simulink library "autolibshared"  (R2019b)
settings: Solver=ode45  StartTime=0.0  StopTime=10.0  RelTol=1e-3  EnableMultiTasking=on
undefined symbols (not defined in the file or in its folder): AccelCycle, aMode, DriveCycle, GearCycle, psi, x_o
libraries: autolibsharedcommon x20, $bdroot x7, autolibutils x2, autolibpowerinfoutils x1
(part 1 of 4)
Description:
  | Automotive Blockset Library: Shared Blocks
settings Model: ModifiedByFormat=The MathWorks, Inc.  Creator=The MathWorks, Inc.  LastModifiedBy=The MathWorks, Inc.
settings SolverCC: MinimalZcImpactIntegration=on
settings DataIOCC: LimitDataPoints=on  SaveFormat=Array  ReturnWorkspaceOutputs=off
settings OptimizationCC: LifeSpan=inf
settings DebuggingCC: SolverPrmCheckMsg=warning  AllowSymbolicDim=off  PregeneratedLibrarySubsystemCodeDiagnostic=none  SFUnexpectedBacktrackingDiag=warning  SFNoUnconditionalDefaultTransitionDiag=warning  SFExecutionAtInitializationDiag=none  ArithmeticOperatorsInVariantConditions=warning
settings ModelReferenceCC: PropagateSignalLabelsOutOfModel=off
settings SFSimCC: SimUseLocalCustomCode=off  CustomCodeUndefinedFunction=UseInterfaceOnly
settings RTWCC: RTWUseLocalCustomCode=off
settings CodeAppCC: StateflowObjectComments=on
settings GRTTargetCC: TargetLangStandard=C89/C90 (ANSI)  GeneratePreprocessorConditionals=Disable all
settings ConfigComp: CovMetricSettings=dw  CovHtmlReporting=on  CovSaveCumulativeToWorkspaceVar=on  CovSaveSingleToWorkspaceVar=on  CovShowResultsExplorer=off  CovExternalEMLEnable=off  CovSFcnEnable=off

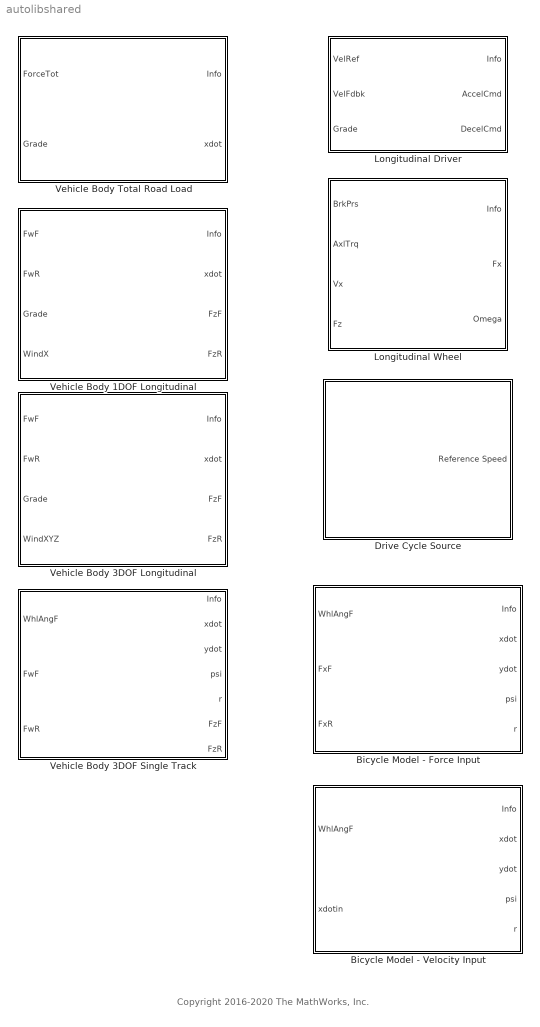
== system autolibshared ==
  note: Copyright 2016-2020 The MathWorks, Inc.
  Bicycle Model - Force Input : Subsystem  mask(Vehicle Body 3DOF Lateral){trackMode=Single (bicycle), inputMode=External longitudinal forces, frontSteerMode=on, rearSteerMode=off, windMode=off, muMode=off, extFMode=off, extMMode=off, aMode=aMode, NF=2, NR=2, m=2000, a=1.4, b=1.6, h=0.35, X_o=0, xdot_o=0, CalphaMode=off, sigmaMode=on, w=[1.4,1.4], Cy_f=12e3, Cy_r=11e3, sigma_f=.1, sigma_r=.1, alpha_f_brk=[-.1 .1], Cy_f_data=[-9e3 9e3], alpha_r_brk=[-.1 .1], Cy_r_data=[-9e3 9e3], Y_o=0, ydot_o=0, Izz=4000, psi_o=0, r_o=0, Af=2, Cd=.3, Cl=.1, Cpm=.1, beta_w=[0:0.01:0.3], Cs=[0:0.03:0.9], Cym=[0:0.01:0.3], Pabs=101325, Tair=273, g=9.81, mu=1, xdot_tol=.01, Fznom=5000, Fxtire_sat=1e6, Fytire_sat=1e6, longOff=0, latOff=0, vertOff=0}
      mask prompts: trackMode "autoblks_shared:autoblkVehBody3DofADTF:blkPrm_trackMode"; inputMode "autoblks_shared:autoblkVehBody3DofADTF:blkPrm_inputMode"; frontSteerMode "autoblks_shared:autoblkVehBody3DofADTF:blkPrm_frontSteerMode"; rearSteerMode "autoblks_shared:autoblkVehBody3DofADTF:blkPrm_rearSteerMode"; windMode "autoblks_shared:autoblkVehBody3DofADTF:blkPrm_windMode"; muMode "autoblks_shared:autoblkVehBody3DofADTF:blkPrm_muMode"; extFMode "autoblks_shared:autoblkVehBody3DofADTF:blkPrm_extFMode"; extMMode "autoblks_shared:autoblkVehBody3DofADTF:blkPrm_extMMode"; NF "autoblks_shared:autoblkVehBody3DofADTF:blkPrm_NF"; NR "autoblks_shared:autoblkVehBody3DofADTF:blkPrm_NR"; m "autoblks_shared:autoblkVehBody3DofADTF:blkPrm_m"; a "autoblks_shared:autoblkVehBody3DofADTF:blkPrm_a"; b "autoblks_shared:autoblkVehBody3DofADTF:blkPrm_b"; h "autoblks_shared:autoblkVehBody3DofADTF:blkPrm_h"; X_o "autoblks_shared:autoblkVehBody3DofADTF:blkPrm_X_o"; xdot_o "autoblks_shared:autoblkVehBody3DofADTF:blkPrm_xdot_o"; CalphaMode "autoblks_shared:autoblkVehBody3DofADTF:blkPrm_CalphaMode"; sigmaMode "autoblks_shared:autoblkVehBody3DofADTF:blkPrm_sigmaMode"; w "autoblks_shared:autoblkVehBody3DofADTF:blkPrm_w"; Cy_f "autoblks_shared:autoblkVehBody3DofADTF:blkPrm_Cy_f"; Cy_r "autoblks_shared:autoblkVehBody3DofADTF:blkPrm_Cy_r"; sigma_f "autoblks_shared:autoblkVehBody3DofADTF:blkPrm_sigma_f"; sigma_r "autoblks_shared:autoblkVehBody3DofADTF:blkPrm_sigma_r"; alpha_f_brk "autoblks_shared:autoblkVehBody3DofADTF:blkPrm_alpha_f_brk"; Cy_f_data "autoblks_shared:autoblkVehBody3DofADTF:blkPrm_Cy_f_data"; alpha_r_brk "autoblks_shared:autoblkVehBody3DofADTF:blkPrm_alpha_r_brk"; Cy_r_data "autoblks_shared:autoblkVehBody3DofADTF:blkPrm_Cy_r_data"; Y_o "autoblks_shared:autoblkVehBody3DofADTF:blkPrm_Y_o"; ydot_o "autoblks_shared:autoblkVehBody3DofADTF:blkPrm_ydot_o"; Izz "autoblks_shared:autoblkVehBody3DofADTF:blkPrm_Izz"; psi_o "autoblks_shared:autoblkVehBody3DofADTF:blkPrm_psi_o"; r_o "autoblks_shared:autoblkVehBody3DofADTF:blkPrm_r_o"; Af "autoblks_shared:autoblkVehBody3DofADTF:blkPrm_Af"; Cd "autoblks_shared:autoblkVehBody3DofADTF:blkPrm_Cd"; Cl "autoblks_shared:autoblkVehBody3DofADTF:blkPrm_Cl"; Cpm "autoblks_shared:autoblkVehBody3DofADTF:blkPrm_Cpm"; beta_w "autoblks_shared:autoblkVehBody3DofADTF:blkPrm_beta_w"; Cs "autoblks_shared:autoblkVehBody3DofADTF:blkPrm_Cs"; Cym "autoblks_shared:autoblkVehBody3DofADTF:blkPrm_Cym"; Pabs "autoblks_shared:autoblkVehBody3DofADTF:blkPrm_Pabs"; Tair "autoblks_shared:autoblkVehBody3DofADTF:blkPrm_Tair"; g "autoblks_shared:autoblkVehBody3DofADTF:blkPrm_g"; mu "autoblks_shared:autoblkVehBody3DofADTF:blkPrm_mu"; xdot_tol "autoblks_shared:autoblkVehBody3DofADTF:blkPrm_xdot_tol"; Fznom "autoblks_shared:autoblkVehBody3DofADTF:blkPrm_Fznom"; Fxtire_sat "autoblks_shared:autoblkVehBody3DofADTF:blkPrm_Fxtire_sat"; Fytire_sat "autoblks_shared:autoblkVehBody3DofADTF:blkPrm_Fytire_sat"; longOff "autoblks_shared:autoblkVehBody3DofADTF:blkPrm_longOff"; latOff "autoblks_shared:autoblkVehBody3DofADTF:blkPrm_latOff"; vertOff "autoblks_shared:autoblkVehBody3DofADTF:blkPrm_vertOff"
      mask help: autoblks_shared:autoblkVehBody3DofADTF:blkDesc
      mask init:
      | [~]=autosharedicon('autolibvehdyn3doflatr',gcb,0);
      mask Help: eval('autosharedhelp(''vbbicycle'')');
      mask TypeOptions trackMode: autoblks_shared:autoblkVehBody3DofADTF:blkCmb_trackMode_c1 | autoblks_shared:autoblkVehBody3DofADTF:blkCmb_trackMode_c2
      mask Callback trackMode: %[~]=vehdynicon('vehdynliblat3dof',gcb,5);
      mask TypeOptions inputMode: autoblks_shared:autoblkVehBody3DofADTF:blkCmb_inputMode_c1 | autoblks_shared:autoblkVehBody3DofADTF:blkCmb_inputMode_c2 | autoblks_shared:autoblkVehBody3DofADTF:blkCmb_inputMode_c3
      mask Callback inputMode: %[~]=vehdynicon('vehdynliblat3dof',gcb,1);
      mask Callback muMode: %[~]=vehdynicon('vehdynliblat3dof',gcb,2);
      mask Callback CalphaMode: %[~]=vehdynicon('vehdynliblat3dof',gcb,3);
      mask Callback sigmaMode: %[~]=vehdynicon('vehdynliblat3dof',gcb,4);
      mask TypeOptions longOff: Vehicle Body 3DOF Single Track/longOff
      mask TypeOptions latOff: Vehicle Body 3DOF Single Track/latOff
      mask TypeOptions vertOff: Vehicle Body 3DOF Single Track/vertOff
      mask DialogControl blockConfig Prompt: autoblks_shared:autoblkVehBody3DofADTF:blkDlg_blockConfig
      mask DialogControl trackMode Prompt: Vehicle track:
      mask DialogControl inputMode Prompt: Axle forces:
      mask DialogControl frontSteerMode Prompt: Front wheel steering
      mask DialogControl rearSteerMode Prompt: Rear wheel steering
      mask DialogControl windMode Prompt: External wind
      mask DialogControl muMode Prompt: External friction
      mask DialogControl extFMode Prompt: External forces
      mask DialogControl extMMode Prompt: External moments
      mask DialogControl ParameterGroupVar Prompt: autoblks_shared:autoblkVehBody3DofADTF:blkDlg_ParameterGroupVar
      mask DialogControl LongPanel Prompt: autoblks_shared:autoblkVehBody3DofADTF:blkDlg_LongPanel
      mask DialogControl NF Prompt: Number of wheels on front axle, NF [-]:
      mask DialogControl NR Prompt: Number of wheels on rear axle, NR [-]:
      mask DialogControl m Prompt: Vehicle mass, m [kg]:
      mask DialogControl a Prompt: Longitudinal distance from center of mass to front axle, a [m]:
      mask DialogControl b Prompt: Longitudinal distance from center of mass to rear axle, b [m]:
      mask DialogControl h Prompt: Vertical distance from center of mass to axle plane, h [m]:
      mask DialogControl X_o Prompt: Initial inertial frame longitudinal position, X_o [m]:
      mask DialogControl xdot_o Prompt: Initial longitudinal velocity, xdot_o [m/s]:
      mask DialogControl LatPanel Prompt: autoblks_shared:autoblkVehBody3DofADTF:blkDlg_LatPanel
      mask DialogControl CalphaMode Prompt: Mapped corner stiffness:
      mask DialogControl sigmaMode Prompt: Include relaxation length dynamics:
      mask DialogControl w Prompt: Track width, w [m]:
      mask DialogControl Cy_f Prompt: Front tire corner stiffness, Cy_f [N/rad]:
      mask DialogControl Cy_r Prompt: Rear tire axle corner stiffness, Cy_r [N/rad]:
      mask DialogControl sigma_f Prompt: Front tire(s) relaxation length, sigma_f [m]:
      mask DialogControl sigma_r Prompt: Rear tire(s) relaxation length, sigma_r [m]:
      mask DialogControl alpha_f_brk Prompt: Front axle slip angle breakpoints, alpha_f_brk [rad]:
      mask DialogControl Cy_f_data Prompt: Front axle corner data, Cy_f_data [N/rad]:
      mask DialogControl alpha_r_brk Prompt: Rear axle slip angle breakpoints, alpha_r_brk [rad]:
      mask DialogControl Cy_r_data Prompt: Rear axle corner data, Cy_r_data [N/rad]:
      mask DialogControl Y_o Prompt: Initial inertial frame lateral displacement, Y_o [m]:
      mask DialogControl ydot_o Prompt: Initial lateral velocity, ydot_o [m/s]:
      mask DialogControl YawPanel Prompt: autoblks_shared:autoblkVehBody3DofADTF:blkDlg_YawPanel
      mask DialogControl Izz Prompt: Yaw polar inertia, Izz [kg*m^2]:
      mask DialogControl psi_o Prompt: Initial yaw angle, psi_o [rad]:
      mask DialogControl r_o Prompt: Initial yaw rate, r_o [rad/s]:
      mask DialogControl AeroParams Prompt: autoblks_shared:autoblkVehBody3DofADTF:blkDlg_AeroParams
      mask DialogControl Af Prompt: Longitudinal drag area, Af [m^2]:
      mask DialogControl Cd Prompt: Longitudinal drag coefficient, Cd [-]:
      mask DialogControl Cl Prompt: Longitudinal lift coefficient, Cl [-]:
      mask DialogControl Cpm Prompt: Longitudinal drag pitch moment, Cpm [-]:
      mask DialogControl beta_w Prompt: Relative wind angle vector, beta_w [rad]:
      mask DialogControl Cs Prompt: Side force coefficient vector, Cs [-]:
      mask DialogControl Cym Prompt: Yaw moment coefficient vector, Cym [-]:
      mask DialogControl EnviroPanel Prompt: autoblks_shared:autoblkVehBody3DofADTF:blkDlg_EnviroPanel
      mask DialogControl Pabs Prompt: Absolute pressure, Pabs [Pa]:
      mask DialogControl Tair Prompt: Air temperature, Tair [K]:
      mask DialogControl g Prompt: Gravitational acceleration, g [m/s^2]:
      mask DialogControl mu Prompt: Nominal friction scaling factor, mu [-]:
      mask DialogControl SimPanel Prompt: autoblks_shared:autoblkVehBody3DofADTF:blkDlg_SimPanel
      mask DialogControl xdot_tol Prompt: Longitudinal velocity tolerance, xdot_tol [m/s]:
      mask DialogControl Fznom Prompt: Nominal normal force, Fznom [N]:
      mask DialogControl Fxtire_sat Prompt: Longitudinal force limit, Fxtire_sat [N]:
      mask DialogControl Fytire_sat Prompt: Lateral force limit, Fytire_sat [N]:
      mask DialogControl longOff Prompt: Geometric longitudinal offset from axle plane, longOff [m]:
      mask DialogControl latOff Prompt: Geometric lateral offset from axle plane, latOff [m]:
      mask DialogControl vertOff Prompt: Geometric vertical offset from axle plane, vertOff [m]:
      mask Display:
      | try
      |     IconInfo = autosharedicon('autolibvehdyn3doflatr',gcb,8);
      | 
      |     image(IconInfo.image, IconInfo.position);
      | 
      |     for i = 1:numel(IconInfo.lconn)
      |         port_label('lconn', i, IconInfo.lconn{i})
      |     end
      | 
      |     for j = 1:numel(IconInfo.rconn)
      |         port_label('rconn', j, IconInfo.rconn{j})
      |     end
      | 
      |     for k = 1:numel(IconInfo.input)
      |         port_label('input', k, IconInfo.input{k})
      |     end
      | 
      |     for m = 1:numel(IconInfo.output)
      |         port_label('output', m, IconInfo.output{m})
      |     end
      | catch
      |     fprintf('Vehicle Body \n 3DOF Lateral')
      | end
  Bicycle Model - Velocity Input : Subsystem  mask(Vehicle Body 3DOF Lateral){trackMode=Single (bicycle), inputMode=External longitudinal velocity, frontSteerMode=on, rearSteerMode=off, windMode=off, muMode=off, extFMode=off, extMMode=off, aMode=aMode, NF=2, NR=2, m=2000, a=1.4, b=1.6, h=0.35, X_o=0, xdot_o=0, CalphaMode=off, sigmaMode=on, w=[1.4,1.4], Cy_f=12e3, Cy_r=11e3, sigma_f=.1, sigma_r=.1, alpha_f_brk=[-.1 .1], Cy_f_data=[-9e3 9e3], alpha_r_brk=[-.1 .1], Cy_r_data=[-9e3 9e3], Y_o=0, ydot_o=0, Izz=4000, psi_o=0, r_o=0, Af=2, Cd=.3, Cl=.1, Cpm=.1, beta_w=[0:0.01:0.3], Cs=[0:0.03:0.9], Cym=[0:0.01:0.3], Pabs=101325, Tair=273, g=9.81, mu=1, xdot_tol=.01, Fznom=5000, Fxtire_sat=1e6, Fytire_sat=1e6, longOff=0, latOff=0, vertOff=0}
      mask prompts: trackMode "autoblks_shared:autoblkVehBody3DofADTx:blkPrm_trackMode"; inputMode "autoblks_shared:autoblkVehBody3DofADTx:blkPrm_inputMode"; frontSteerMode "autoblks_shared:autoblkVehBody3DofADTx:blkPrm_frontSteerMode"; rearSteerMode "autoblks_shared:autoblkVehBody3DofADTx:blkPrm_rearSteerMode"; windMode "autoblks_shared:autoblkVehBody3DofADTx:blkPrm_windMode"; muMode "autoblks_shared:autoblkVehBody3DofADTx:blkPrm_muMode"; extFMode "autoblks_shared:autoblkVehBody3DofADTx:blkPrm_extFMode"; extMMode "autoblks_shared:autoblkVehBody3DofADTx:blkPrm_extMMode"; NF "autoblks_shared:autoblkVehBody3DofADTx:blkPrm_NF"; NR "autoblks_shared:autoblkVehBody3DofADTx:blkPrm_NR"; m "autoblks_shared:autoblkVehBody3DofADTx:blkPrm_m"; a "autoblks_shared:autoblkVehBody3DofADTx:blkPrm_a"; b "autoblks_shared:autoblkVehBody3DofADTx:blkPrm_b"; h "autoblks_shared:autoblkVehBody3DofADTx:blkPrm_h"; X_o "autoblks_shared:autoblkVehBody3DofADTx:blkPrm_X_o"; xdot_o "autoblks_shared:autoblkVehBody3DofADTx:blkPrm_xdot_o"; CalphaMode "autoblks_shared:autoblkVehBody3DofADTx:blkPrm_CalphaMode"; sigmaMode "autoblks_shared:autoblkVehBody3DofADTx:blkPrm_sigmaMode"; w "autoblks_shared:autoblkVehBody3DofADTx:blkPrm_w"; Cy_f "autoblks_shared:autoblkVehBody3DofADTx:blkPrm_Cy_f"; Cy_r "autoblks_shared:autoblkVehBody3DofADTx:blkPrm_Cy_r"; sigma_f "autoblks_shared:autoblkVehBody3DofADTx:blkPrm_sigma_f"; sigma_r "autoblks_shared:autoblkVehBody3DofADTx:blkPrm_sigma_r"; alpha_f_brk "autoblks_shared:autoblkVehBody3DofADTx:blkPrm_alpha_f_brk"; Cy_f_data "autoblks_shared:autoblkVehBody3DofADTx:blkPrm_Cy_f_data"; alpha_r_brk "autoblks_shared:autoblkVehBody3DofADTx:blkPrm_alpha_r_brk"; Cy_r_data "autoblks_shared:autoblkVehBody3DofADTx:blkPrm_Cy_r_data"; Y_o "autoblks_shared:autoblkVehBody3DofADTx:blkPrm_Y_o"; ydot_o "autoblks_shared:autoblkVehBody3DofADTx:blkPrm_ydot_o"; Izz "autoblks_shared:autoblkVehBody3DofADTx:blkPrm_Izz"; psi_o "autoblks_shared:autoblkVehBody3DofADTx:blkPrm_psi_o"; r_o "autoblks_shared:autoblkVehBody3DofADTx:blkPrm_r_o"; Af "autoblks_shared:autoblkVehBody3DofADTx:blkPrm_Af"; Cd "autoblks_shared:autoblkVehBody3DofADTx:blkPrm_Cd"; Cl "autoblks_shared:autoblkVehBody3DofADTx:blkPrm_Cl"; Cpm "autoblks_shared:autoblkVehBody3DofADTx:blkPrm_Cpm"; beta_w "autoblks_shared:autoblkVehBody3DofADTx:blkPrm_beta_w"; Cs "autoblks_shared:autoblkVehBody3DofADTx:blkPrm_Cs"; Cym "autoblks_shared:autoblkVehBody3DofADTx:blkPrm_Cym"; Pabs "autoblks_shared:autoblkVehBody3DofADTx:blkPrm_Pabs"; Tair "autoblks_shared:autoblkVehBody3DofADTx:blkPrm_Tair"; g "autoblks_shared:autoblkVehBody3DofADTx:blkPrm_g"; mu "autoblks_shared:autoblkVehBody3DofADTx:blkPrm_mu"; xdot_tol "autoblks_shared:autoblkVehBody3DofADTx:blkPrm_xdot_tol"; Fznom "autoblks_shared:autoblkVehBody3DofADTx:blkPrm_Fznom"; Fxtire_sat "autoblks_shared:autoblkVehBody3DofADTx:blkPrm_Fxtire_sat"; Fytire_sat "autoblks_shared:autoblkVehBody3DofADTx:blkPrm_Fytire_sat"; longOff "autoblks_shared:autoblkVehBody3DofADTx:blkPrm_longOff"; latOff "autoblks_shared:autoblkVehBody3DofADTx:blkPrm_latOff"; vertOff "autoblks_shared:autoblkVehBody3DofADTx:blkPrm_vertOff"
      mask help: autoblks_shared:autoblkVehBody3DofADTx:blkDesc
      mask init:
      | [~]=autosharedicon('autolibvehdyn3doflatr',gcb,0);
      mask Help: eval('autosharedhelp(''vbbicycle'')');
      mask TypeOptions trackMode: autoblks_shared:autoblkVehBody3DofADTx:blkCmb_trackMode_c1 | autoblks_shared:autoblkVehBody3DofADTx:blkCmb_trackMode_c2
      mask Callback trackMode: %[~]=vehdynicon('vehdynliblat3dof',gcb,5);
      mask TypeOptions inputMode: autoblks_shared:autoblkVehBody3DofADTx:blkCmb_inputMode_c1 | autoblks_shared:autoblkVehBody3DofADTx:blkCmb_inputMode_c2 | autoblks_shared:autoblkVehBody3DofADTx:blkCmb_inputMode_c3
      mask Callback inputMode: %[~]=vehdynicon('vehdynliblat3dof',gcb,1);
      mask Callback muMode: %[~]=vehdynicon('vehdynliblat3dof',gcb,2);
      mask Callback CalphaMode: %[~]=vehdynicon('vehdynliblat3dof',gcb,3);
      mask Callback sigmaMode: %[~]=vehdynicon('vehdynliblat3dof',gcb,4);
      mask TypeOptions longOff: Vehicle Body 3DOF Single Track/longOff
      mask TypeOptions latOff: Vehicle Body 3DOF Single Track/latOff
      mask TypeOptions vertOff: Vehicle Body 3DOF Single Track/vertOff
      mask DialogControl blockConfig Prompt: autoblks_shared:autoblkVehBody3DofADTx:blkDlg_blockConfig
      mask DialogControl trackMode Prompt: Vehicle track:
      mask DialogControl inputMode Prompt: Axle forces:
      mask DialogControl frontSteerMode Prompt: Front wheel steering
      mask DialogControl rearSteerMode Prompt: Rear wheel steering
      mask DialogControl windMode Prompt: External wind
      mask DialogControl muMode Prompt: External friction
      mask DialogControl extFMode Prompt: External forces
      mask DialogControl extMMode Prompt: External moments
      mask DialogControl ParameterGroupVar Prompt: autoblks_shared:autoblkVehBody3DofADTx:blkDlg_ParameterGroupVar
      mask DialogControl LongPanel Prompt: autoblks_shared:autoblkVehBody3DofADTx:blkDlg_LongPanel
      mask DialogControl NF Prompt: Number of wheels on front axle, NF [-]:
      mask DialogControl NR Prompt: Number of wheels on rear axle, NR [-]:
      mask DialogControl m Prompt: Vehicle mass, m [kg]:
      mask DialogControl a Prompt: Longitudinal distance from center of mass to front axle, a [m]:
      mask DialogControl b Prompt: Longitudinal distance from center of mass to rear axle, b [m]:
      mask DialogControl h Prompt: Vertical distance from center of mass to axle plane, h [m]:
      mask DialogControl X_o Prompt: Initial inertial frame longitudinal position, X_o [m]:
      mask DialogControl xdot_o Prompt: Initial longitudinal velocity, xdot_o [m/s]:
      mask DialogControl LatPanel Prompt: autoblks_shared:autoblkVehBody3DofADTx:blkDlg_LatPanel
      mask DialogControl CalphaMode Prompt: Mapped corner stiffness:
      mask DialogControl sigmaMode Prompt: Include relaxation length dynamics:
      mask DialogControl w Prompt: Track width, w [m]:
      mask DialogControl Cy_f Prompt: Front tire corner stiffness, Cy_f [N/rad]:
      mask DialogControl Cy_r Prompt: Rear tire axle corner stiffness, Cy_r [N/rad]:
      mask DialogControl sigma_f Prompt: Front tire(s) relaxation length, sigma_f [m]:
      mask DialogControl sigma_r Prompt: Rear tire(s) relaxation length, sigma_r [m]:
      mask DialogControl alpha_f_brk Prompt: Front axle slip angle breakpoints, alpha_f_brk [rad]:
      mask DialogControl Cy_f_data Prompt: Front axle corner data, Cy_f_data [N/rad]:
      mask DialogControl alpha_r_brk Prompt: Rear axle slip angle breakpoints, alpha_r_brk [rad]:
      mask DialogControl Cy_r_data Prompt: Rear axle corner data, Cy_r_data [N/rad]:
      mask DialogControl Y_o Prompt: Initial inertial frame lateral displacement, Y_o [m]:
      mask DialogControl ydot_o Prompt: Initial lateral velocity, ydot_o [m/s]:
      mask DialogControl YawPanel Prompt: autoblks_shared:autoblkVehBody3DofADTx:blkDlg_YawPanel
      mask DialogControl Izz Prompt: Yaw polar inertia, Izz [kg*m^2]:
      mask DialogControl psi_o Prompt: Initial yaw angle, psi_o [rad]:
      mask DialogControl r_o Prompt: Initial yaw rate, r_o [rad/s]:
      mask DialogControl AeroParams Prompt: autoblks_shared:autoblkVehBody3DofADTx:blkDlg_AeroParams
      mask DialogControl Af Prompt: Longitudinal drag area, Af [m^2]:
      mask DialogControl Cd Prompt: Longitudinal drag coefficient, Cd [-]:
      mask DialogControl Cl Prompt: Longitudinal lift coefficient, Cl [-]:
      mask DialogControl Cpm Prompt: Longitudinal drag pitch moment, Cpm [-]:
      mask DialogControl beta_w Prompt: Relative wind angle vector, beta_w [rad]:
      mask DialogControl Cs Prompt: Side force coefficient vector, Cs [-]:
      mask DialogControl Cym Prompt: Yaw moment coefficient vector, Cym [-]:
      mask DialogControl EnviroPanel Prompt: autoblks_shared:autoblkVehBody3DofADTx:blkDlg_EnviroPanel
      mask DialogControl Pabs Prompt: Absolute pressure, Pabs [Pa]:
      mask DialogControl Tair Prompt: Air temperature, Tair [K]:
      mask DialogControl g Prompt: Gravitational acceleration, g [m/s^2]:
      mask DialogControl mu Prompt: Nominal friction scaling factor, mu [-]:
      mask DialogControl SimPanel Prompt: autoblks_shared:autoblkVehBody3DofADTx:blkDlg_SimPanel
      mask DialogControl xdot_tol Prompt: Longitudinal velocity tolerance, xdot_tol [m/s]:
      mask DialogControl Fznom Prompt: Nominal normal force, Fznom [N]:
      mask DialogControl Fxtire_sat Prompt: Longitudinal force limit, Fxtire_sat [N]:
      mask DialogControl Fytire_sat Prompt: Lateral force limit, Fytire_sat [N]:
      mask DialogControl longOff Prompt: Geometric longitudinal offset from axle plane, longOff [m]:
      mask DialogControl latOff Prompt: Geometric lateral offset from axle plane, latOff [m]:
      mask DialogControl vertOff Prompt: Geometric vertical offset from axle plane, vertOff [m]:
      mask Display:
      | try
      |     IconInfo = autosharedicon('autolibvehdyn3doflatr',gcb,8);
      | 
      |     image(IconInfo.image, IconInfo.position);
      | 
      |     for i = 1:numel(IconInfo.lconn)
      |         port_label('lconn', i, IconInfo.lconn{i})
      |     end
      | 
      |     for j = 1:numel(IconInfo.rconn)
      |         port_label('rconn', j, IconInfo.rconn{j})
      |     end
      | 
      |     for k = 1:numel(IconInfo.input)
      |         port_label('input', k, IconInfo.input{k})
      |     end
      | 
      |     for m = 1:numel(IconInfo.output)
      |         port_label('output', m, IconInfo.output{m})
      |     end
      | catch
      |     fprintf('Vehicle Body \n 3DOF Lateral')
      | end
  Drive Cycle Source : Subsystem  mask(Drive Cycle Source){cycleVar=FTP75, wsVar=, fileVar=cycleFTP75.mat, tfinal=2474  seconds, cycleRepeat=off, outAccPort=off, outGearPort=off, gearList=No gear data, t_wot1=5, xdot_woto=0, xdot_wot1=30, t_wot2=20, xdot_wot2=0, t_wotend=30, srcUnit=m/s, outUnit=m/s, srcAccUnit=m/s/s, outAccUnit=m/s^2, dt=0, aMode=aMode}
      mask prompts: cycleVar "autoblks_shared:autoblkDriveCycleSource:blkPrm_cycleVar"; wsVar "autoblks_shared:autoblkDriveCycleSource:blkPrm_wsVar"; fileVar "autoblks_shared:autoblkDriveCycleSource:blkPrm_fileVar"; tfinal "autoblks_shared:autoblkDriveCycleSource:blkPrm_tfinal"; cycleRepeat "autoblks_shared:autoblkDriveCycleSource:blkPrm_cycleRepeat"; outAccPort "autoblks_shared:autoblkDriveCycleSource:blkPrm_outAccPort"; outGearPort "Output gear shift data"; gearList "Select gear data:"; t_wot1 "autoblks_shared:autoblkDriveCycleSource:blkPrm_t_wot1"; xdot_woto "autoblks_shared:autoblkDriveCycleSource:blkPrm_xdot_woto"; xdot_wot1 "autoblks_shared:autoblkDriveCycleSource:blkPrm_xdot_wot1"; t_wot2 "autoblks_shared:autoblkDriveCycleSource:blkPrm_t_wot2"; xdot_wot2 "autoblks_shared:autoblkDriveCycleSource:blkPrm_xdot_wot2"; t_wotend "autoblks_shared:autoblkDriveCycleSource:blkPrm_t_wotend"; srcUnit "autoblks_shared:autoblkDriveCycleSource:blkPrm_srcUnit"; outUnit "autoblks_shared:autoblkDriveCycleSource:blkPrm_outUnit"; srcAccUnit "autoblks_shared:autoblkDriveCycleSource:blkPrm_srcAccUnit"; outAccUnit "autoblks_shared:autoblkDriveCycleSource:blkPrm_outAccUnit"; dt "autoblks_shared:autoblkDriveCycleSource:blkPrm_dt"
      mask help: autoblks_shared:autoblkDriveCycleSource:blkDesc
      mask init:
      | [DriveCycle, AccelCycle, GearCycle] = autosharedicon('autolibdrivecycle',gcb,0);
      settings: AttributesFormatString=%<cycleVar> (%<tfinal>)
      mask Help: eval('autosharedhelp(''pbdrivecyclelong'')');
      mask TypeOptions cycleVar: FTP72 | FTP75 | US06 | SC03 | HWFET | NYCC | HUDDS | LA92 | LA92Short | IM240 | UDDS | WLTP Class 1 | WLTP Class 2 | WLTP Class 3 | ECE R15 (single cycle) | ECE R15 (four cycles) | EUDC | ECE Extra-Urban Driving Cycle (Low Powered Vehicles) | NEDC | ADAC BAB 130 | Artemis Urban | Artemis Rural Road | Artemis Motorway 130 kmph | Artemis Motorway 150 kmph | JC08 | JC08 Hot | Japanese 10 Mode | Japanese 15 Mode | Japanese 10-15 Mode | World Harmonized Vehicle Cycle (WHVC) | Braunschweig City Driving Cycle | Central Business District (CBD) Cycle | Business Arterial Commuter (BAC) - Arterial Cycle | Business Arterial Commuter (BAC) - Commuter Cycle | City Suburban Heavy Vehicle Cycle (CSC) | Neighborhood Refuse Truck Cycle | New York Composite Cycle | New York Bus Cycle | Manhattan Bus Cycle | Heavy Heavy-Duty Diesel Truck (HHDDT) - Creep Mode | Heavy Heavy-Duty Diesel Truck (HHDDT) - Transient Mode | Heavy Heavy-Duty Diesel Truck (HHDDT) - Cruise Mode | Orange County Bus Cycle | West Virginia University 5-Peak Truck Cycle | RTS 95 | ETC FIGE Version 4 | JE05 Japanese Transient Mode for vehicles > 3500 kg GVW | CUEDC Petrol cycle | CUEDC SPC240 cycle | CUEDC diesel cycle - MC | CUEDC diesel cycle - NA | CUEDC diesel cycle - NB | CUEDC diesel cycle - ME | CUEDC diesel cycle - NC | CUEDC diesel cycle - NCH | Wide Open Throttle (WOT) | Workspace variable | .mat, .xls, .xlsx or .txt file
      mask Callback cycleVar: [~,~] = autosharedicon('autolibdrivecycle',gcb,1);
      mask Callback outAccPort: [~,~] = autosharedicon('autolibdrivecycle',gcb,5);
      mask Callback outGearPort: [~,~] = autosharedicon('autolibdrivecycle',gcb,6);
      mask TypeOptions gearList: No gear data
      mask TypeOptions srcUnit: timing mode/Continuous/Spd/Unit | timing mode/Discrete/Spd/Unit
      mask TypeOptions outUnit: Reference Speed/Unit
      mask TypeOptions srcAccUnit: timing mode/Continuous/Acc/Unit | timing mode/Discrete/Acc/Unit
      mask DialogControl cycleVar Prompt: Drive cycle source:
      mask DialogControl wsVar Prompt: From workspace:
      mask DialogControl fileVar Prompt: Drive cycle source file:
      mask DialogControl wsVarSel Prompt: autoblks_shared:autoblkDriveCycleSource:blkDlg_wsVarSel
      mask DialogControl wsVarSel Callback:
      | set_param(gcb,'cycleVar','Workspace variable');
      | [~,~] = autosharedicon('autolibdrivecycle',gcb,1);
      mask DialogControl fileSel Prompt: autoblks_shared:autoblkDriveCycleSource:blkDlg_fileSel
      mask DialogControl fileSel Callback: [~,~] = autosharedicon('autolibdrivecycle',gcb,2);
      mask DialogControl getData Prompt: autoblks_shared:autoblkDriveCycleSource:blkDlg_getData
      mask DialogControl getData Callback: autoDataPackage(gcb)
      mask DialogControl tfinal Prompt: Total drive cycle time:
      mask DialogControl cycleRepeat Prompt: Repeat cyclically
      mask DialogControl outAccPort Prompt: Output acceleration
      mask DialogControl wotParam Prompt: autoblks_shared:autoblkDriveCycleSource:blkDlg_wotParam
      mask DialogControl t_wot1 Prompt: Start time, t_wot1 [s]:
      mask DialogControl xdot_woto Prompt: Initial reference speed, xdot_woto []:
      mask DialogControl xdot_wot1 Prompt: Nominal reference speed, xdot_wot1 []:
      mask DialogControl t_wot2 Prompt: Time to start deceleration, t_wot2 [s]:
      mask DialogControl xdot_wot2 Prompt: Final reference speed, xdot_wot2 []:
      mask DialogControl t_wotend Prompt: WOT simulation time, t_wotend []:
      mask DialogControl unitsParam Prompt: autoblks_shared:autoblkDriveCycleSource:blkDlg_unitsParam
      mask DialogControl srcUnit Prompt: Source velocity units (e.g., m/s, km/h, mph):
      mask DialogControl outUnit Prompt: Output velocity units (e.g., m/s, km/h, mph):
      mask DialogControl srcAccUnit Prompt: Source acceleration units (e.g., m/s^2, ft/s^2):
      mask DialogControl outAccUnit Prompt: Output acceleration units (e.g., m/s^2, ft/s^2):
      mask DialogControl dt Prompt: Output sample period (0 for continuous), dt [s]:
      mask DialogControl updateSim Prompt: autoblks_shared:autoblkDriveCycleSource:blkDlg_updateSim
      mask DialogControl updateSim Callback: [~,~] = autosharedicon('autolibdrivecycle',gcb,3);
      mask DialogControl plotCycle Prompt: autoblks_shared:autoblkDriveCycleSource:blkDlg_plotCycle
      mask DialogControl plotCycle Callback: [~,~] = autosharedicon('autolibdrivecycle',gcb,4);
      mask Display:
      | try
      |     if exist('DriveCycle','var') && ~isempty(DriveCycle)
      |         plot(DriveCycle.Time./max(DriveCycle.Time).*0.75,DriveCycle.Data./max(DriveCycle.Data))
      |     end
      |     AliasNames = {'Reference Speed','RefSpd';...
      |                   'Reference Accel','RefAcc';...
      |                   'Reference Gear','RefGear'};
      |     IconInfo = autoblksgetportlabels(gcb, AliasNames);
      |     for m = 1:numel(IconInfo.output)
      |         port_label('output', m, IconInfo.output{m})
      |     end
      | catch
      |     fprintf('Drive Cycle Source')
      | end
  Longitudinal Driver : Subsystem  SystemSampleTime=.01  mask(Longitudinal Driver){cntrlType=PI, shftType=None, velUnits=m/s, gearOut=off, Kp=10, Ki=5, Kff=.1, Kg=0, VehVelVec=[0 100], KffVec=[.1 .1], KpVec=[10 10], KiVec=[5 5], KgVec=[0 0], m=1500, Kpt=10000, tau=.2, L=4, aR=200, bR=2.5, cR=.5, g=9.81, vnom=5, Kaw=1, tauerr=.01, tauPt=2, GearInit=0, tShift=.1, pdlVec=[0.1 0.4 0.5 0.9], upShftTbl=[-1 12.9375 26.4375 39.9375 51.18749999999999 62.4375 72.84375 83.25;-1 16.3125 29.8125 43.3125 54.5624 65.8125 76.78125 87.75;-1 19.6875 33.1875 46.68749999999999 57.9375 69.1875 80.71875 92.25;-1 33 52.5 77.25 100.5 138.75 161.875 185], dwnShftTbl=[1 9.5625 23.0625 36.5625 47.8125 59.0625 68.90625 78.75;1 12.9375 26.4375 39.9375 51.18749999999999 62.4375 72.84375 83.25;1 16.3125 29.8125 43.3125 54.562499 65.8125 76.78125 87.75;1 19.6875 33.1875 46.68749999999999 57.9375 69.1875 80.71875 92.25], tClutch=.5, tRev=.5, tPark=120, aMode=aMode, UpGearVec=[0  1  2  3  4  5  6  7], DownGearVec=[1  2  3  4  5  6  7  8]}
      mask prompts: cntrlType "autoblks_shared:autoblkLongitudinalDriver:blkPrm_cntrlType"; shftType "autoblks_shared:autoblkLongitudinalDriver:blkPrm_shftType"; velUnits "autoblks_shared:autoblkLongitudinalDriver:blkPrm_velUnits"; gearOut "autoblks_shared:autoblkLongitudinalDriver:blkPrm_gearOut"; Kp "autoblks_shared:autoblkLongitudinalDriver:blkPrm_Kp"; Ki "autoblks_shared:autoblkLongitudinalDriver:blkPrm_Ki"; Kff "autoblks_shared:autoblkLongitudinalDriver:blkPrm_Kff"; Kg "autoblks_shared:autoblkLongitudinalDriver:blkPrm_Kg"; VehVelVec "autoblks_shared:autoblkLongitudinalDriver:blkPrm_VehVelVec"; KffVec "autoblks_shared:autoblkLongitudinalDriver:blkPrm_KffVec"; KpVec "autoblks_shared:autoblkLongitudinalDriver:blkPrm_KpVec"; KiVec "autoblks_shared:autoblkLongitudinalDriver:blkPrm_KiVec"; KgVec "autoblks_shared:autoblkLongitudinalDriver:blkPrm_KgVec"; m "autoblks_shared:autoblkLongitudinalDriver:blkPrm_m"; Kpt "autoblks_shared:autoblkLongitudinalDriver:blkPrm_Kpt"; tau "autoblks_shared:autoblkLongitudinalDriver:blkPrm_tau"; L "autoblks_shared:autoblkLongitudinalDriver:blkPrm_L"; aR "autoblks_shared:autoblkLongitudinalDriver:blkPrm_aR"; bR "autoblks_shared:autoblkLongitudinalDriver:blkPrm_bR"; cR "autoblks_shared:autoblkLongitudinalDriver:blkPrm_cR"; g "autoblks_shared:autoblkLongitudinalDriver:blkPrm_g"; vnom "autoblks_shared:autoblkLongitudinalDriver:blkPrm_vnom"; Kaw "autoblks_shared:autoblkLongitudinalDriver:blkPrm_Kaw"; tauerr "autoblks_shared:autoblkLongitudinalDriver:blkPrm_tauerr"; tauPt "Powertrain time constant, tauPt [s]:"; GearInit "autoblks_shared:autoblkLongitudinalDriver:blkPrm_GearInit"; tShift "autoblks_shared:autoblkLongitudinalDriver:blkPrm_tShift"; pdlVec "autoblks_shared:autoblkLongitudinalDriver:blkPrm_pdlVec"; upShftTbl "autoblks_shared:autoblkLongitudinalDriver:blkPrm_upShftTbl"; dwnShftTbl "autoblks_shared:autoblkLongitudinalDriver:blkPrm_dwnShftTbl"; tClutch "autoblks_shared:autoblkLongitudinalDriver:blkPrm_tClutch"; tRev "autoblks_shared:autoblkLongitudinalDriver:blkPrm_tRev"; tPark "autoblks_shared:autoblkLongitudinalDriver:blkPrm_tPark"; UpGearVec "autoblks_shared:autoblkLongitudinalDriver:blkPrm_UpGearVec"; DownGearVec "autoblks_shared:autoblkLongitudinalDriver:blkPrm_DownGearVec"
      mask help: autoblks_shared:autoblkLongitudinalDriver:blkDesc
      mask init:
      | [~]=autosharedicon('autoliboperlong',gcb,0);
      mask Help: eval('autosharedhelp(''pbopmodlong'')');
      mask TypeOptions cntrlType: autoblks_shared:autoblkLongitudinalDriver:blkCmb_cntrlType_c1 | autoblks_shared:autoblkLongitudinalDriver:blkCmb_cntrlType_c2 | autoblks_shared:autoblkLongitudinalDriver:blkCmb_cntrlType_c3
      mask Callback cntrlType: [~]=autosharedicon('autoliboperlong',gcb,1);
      mask TypeOptions shftType: Longitudinal Driver/shftType
      mask TypeOptions velUnits: VelRef/Unit
      mask Callback velUnits: [~]=autosharedicon('autoliboperlong',gcb,1);
      mask DialogControl modeConfig Prompt: autoblks_shared:autoblkLongitudinalDriver:blkDlg_modeConfig
      mask DialogControl cntrlType Prompt: Control type, cntrlType:
      mask DialogControl shftType Prompt: Shift type, shftType:
      mask DialogControl velUnits Prompt: Reference and feedback units, velUnits :
      mask DialogControl gearOut Prompt: Output gear signal
      mask DialogControl CntrlParamPanel Prompt: autoblks_shared:autoblkLongitudinalDriver:blkDlg_CntrlParamPanel
      mask DialogControl PIParam Prompt: autoblks_shared:autoblkLongitudinalDriver:blkDlg_PIParam
      mask DialogControl Kp Prompt: Proportional gain, Kp []:
      mask DialogControl Ki Prompt: Integral gain, Ki []:
      mask DialogControl Kff Prompt: Velocity feed-forward, Kff []:
      mask DialogControl Kg Prompt: Grade feed-forward, Kg [1/deg]:
      mask DialogControl PISchedParam Prompt: autoblks_shared:autoblkLongitudinalDriver:blkDlg_PISchedParam
      mask DialogControl VehVelVec Prompt: Velocity gain breakpoints, VehVelVec:
      mask DialogControl KffVec Prompt: Velocity feed-forward gain values, KffVec []:
      mask DialogControl KpVec Prompt: Proportional gain values, KpVec []:
      mask DialogControl KiVec Prompt: Integral gain values, KiVec []:
      mask DialogControl KgVec Prompt: Grade feed-forward values, KgVec [1/deg]:
      mask DialogControl PredParam Prompt: autoblks_shared:autoblkLongitudinalDriver:blkDlg_PredParam
      mask DialogControl m Prompt: Vehicle mass, m [kg]:
      mask DialogControl Kpt Prompt: Effective vehicle total tractive force, Kpt [N]:
      mask DialogControl tau Prompt: Driver response time, tau [s]:
      mask DialogControl L Prompt: Preview distance, L [m]:
      mask DialogControl aR Prompt: Rolling resistance coefficient, aR [N]:
      mask DialogControl bR Prompt: Rolling and driveline resistance coefficient, bR [N*s/m]:
      mask DialogControl cR Prompt: Aerodynamic drag coefficient, cR [N*s^2/m^2]:
      mask DialogControl g Prompt: Gravitational constant, g [m/s^2]:
      mask DialogControl vnom Prompt: Nominal speed, vnom [velUnits]:
      mask DialogControl Kaw Prompt: Anti-windup, Kaw []:
      mask DialogControl tauerr Prompt: Error filter time constant, tauerr [s]:
      mask DialogControl shiftParamPanel Prompt: autoblks_shared:autoblkLongitudinalDriver:blkDlg_shiftParamPanel
      mask DialogControl GearInit Prompt: Initial gear, GearInit []:
      mask DialogControl tShift Prompt: Time required to shift, tShift [s]:
      mask DialogControl pdlVec Prompt: Up and down shift accelerator pedal positions, pdlVec []:
      mask DialogControl upShftTbl Prompt: Upshift velocity data table, upShftTbl [velUnits]:
      mask DialogControl dwnShftTbl Prompt: Downshift velocity data table, dwnShftTbl [velUnits]:
      mask DialogControl tClutch Prompt: Time required to shift, tClutch [s]:
      mask DialogControl tRev Prompt: Time required to engage reverse from neutral, tRev [s]:
      mask DialogControl tPark Prompt: Time required to engage park from neutral, tPark [s]:
      mask DialogControl UpGearVec Prompt: Upshift gear vector, UpGearVec []:
      mask DialogControl DownGearVec Prompt: Downshift gear vector, DownGearVec []:
      mask Display:
      | try
      |     IconInfo = autosharedicon('autoliboperlong', gcb, 4);
      | 
      |     image(IconInfo.image, IconInfo.position);
      | 
      |     for i = 1:numel(IconInfo.lconn)
      |         port_label('lconn', i, IconInfo.lconn{i})
      |     end
      | 
      |     for j = 1:numel(IconInfo.rconn)
      |         port_label('rconn', j, IconInfo.rconn{j})
      |     end
      | 
      |     for k = 1:numel(IconInfo.input)
      |         port_label('input', k, IconInfo.input{k})
      |     end
      | 
      |     for m = 1:numel(IconInfo.output)
      |         port_label('output', m, IconInfo.output{m})
      |     end
      | catch
      |     fprintf('Longitudinal \n Driver')
      | end
  Longitudinal Wheel : Subsystem  mask(Longitudinal Wheel){FxType=Magic Formula constant value, rollingType=None, BrakeType=Disc, vertType=None, lam_x=1, extMu=off, aMode=aMode, br=0.001, Iyy=0.8, omegao=0, Lrel=0.5, Re=0.3, UNLOADED_RADIUS=0.4, LONGVL=16, gamma=0, NOMPRES=220000, press=220000, extPress=off, Dx=1, Cx=1.65, Bx=10, Ex=0.01, PCX1=1.6, PDX1=1, PDX2=-0.08, PDX3=0, PEX1=0.112, PEX2=0.313, PEX3=0, PEX4=0.0016, PKX1=21.7, PKX2=13.77, PKX3=-0.412, PHX1=2.1585E-4, PHX2=0.00115, PVX1=1.5973E-5, PVX2=1.043E-4, PPX1=-0.3489, PPX2=0.382, PPX3=-0.09634, PPX4=0.06447, lam_muV=1, lam_Kxkappa=1, lam_Cx=1, lam_Ex=0, lam_Hx=1, lam_Vx=1, kappaFx=[-1,-0.78476,-0.61585,-0.48329,-0.37927,-0.29764,-0.23357,-0.1833,-0.14384,-0.11288,-0.088587,-0.069519,-0.054556,-0.042813,-0.033598,-0.026367,-0.020691,-0.016238,-0.012743,-0.01,0.01,0.012743,0.016238,0.020691,0.026367,0.033598,0.042813,0.054556,0.069519,0.088587,0.11288,0.14384,0.1833,0.23357,0.29764,0.37927,0.48329,0.61585,0.78476,1], FzFx=[0,200,400,600,800,1000,1200,1400,1600,1800,2000,2200,2400,2600,2800,3000,3200,3400,3600,3800,4000,4200,4400,4600,4800,5000,5200,5400,5600,5800,6000,6200,6400,6600,6800,7000,7200,7400,7600,7800,8000,8200,8400,8600,8800,9000,9200,9400,9600,9800,10000], FxMap=[-0,-131.22,-262.44,-393.66,-524.88,-656.1,-787.32,-918.54,-1049.8,-1181,-1312.2,-1443.4,-1574.6,-1705.9,-1837.1,-1968.3,-2099.5,-2230.7,-2362,-2493.2,-2624.4,-2755.6,-2886.8,-3018.1,-3149.3,-3280.5,-3411.7,-3542.9,-3674.2,-3805.4,-3936.6,-4067.8,-4199,-4330.2,-4461.5,-4592.7,-4723.9,-4855.1,-4986.3,-5117.6,-5248.8,-5380,-5511.2,-5642.4,-5773.7,-5904.9,-6036.1,-6167.3,-6298.5,-6429.8,-6561 -0,-137.87,-275.75,-413.62,-551.49,-689.36,-827.24,-965.11,-1103,-1240.9,-1378.7,-1516.6,-1654.5,-1792.3,-1930.2,-2068.1,-2206,-2343.8,-2481.7,-2619.6,-2757.5,-2895.3,-3033.2,-3171.1,-3308.9,-3446.8,-3584.7,-3722.6,-3860.4,-3998.3,-4136.2,-4274,-4411.9,-4549.8,-4687.7,-4825.5,-4963.4,-5101.3,-5239.2,-5377,-5514.9,-5652.8,-5790.6,-5928.5,-6066.4,-6204.3,-6342.1,-6480,-6617.9,-6755.8,-6893.6 -0,-145.88,-291.75,-437.63,-583.5,-729.38,-875.25,-1021.1,-1167,-1312.9,-1458.8,-1604.6,-1750.5,-1896.4,-2042.3,-2188.1,-2334,-2479.9,-2625.8,-2771.6,-2917.5,-3063.4,-3209.3,-3355.1,-3501,-3646.9,-3792.8,-3938.6,-4084.5,-4230.4,-4376.3,-4522.1,-4668,-4813.9,-4959.8,-5105.6,-5251.5,-5397.4,-5543.3,-5689.1,-5835,-5980.9,-6126.8,-6272.6,-6418.5,-6564.4,-6710.3,-6856.1,-7002,-7147.9,-7293.8 -0,-155.26,-310.53,-465.79,-621.05,-776.32,-931.58,-1086.8,-1242.1,-1397.4,-1552.6,-1707.9,-1863.2,-2018.4,-2173.7,-2328.9,-2484.2,-2639.5,-2794.7,-2950,-3105.3,-3260.5,-3415.8,-3571.1,-3726.3,-3881.6,-4036.8,-4192.1,-4347.4,-4502.6,-4657.9,-4813.2,-4968.4,-5123.7,-5278.9,-5434.2,-5589.5,-5744.7,-5900,-6055.3,-6210.5,-6365.8,-6521.1,-6676.3,-6831.6,-6986.8,-7142.1,-7297.4,-7452.6,-7607.9,-7763.2 -0,-165.86,-331.71,-497.57,-663.43,-829.28,-995.14,-1161,-1326.9,-1492.7,-1658.6,-1824.4,-1990.3,-2156.1,-2322,-2487.8,-2653.7,-2819.6,-2985.4,-3151.3,-3317.1,-3483,-3648.8,-3814.7,-3980.6,-4146.4,-4312.3,-4478.1,-4644,-4809.8,-4975.7,-5141.5,-5307.4,-5473.3,-5639.1,-5805,-5970.8,-6136.7,-6302.5,-6468.4,-6634.3,-6800.1,-6966,-7131.8,-7297.7,-7463.5,-7629.4,-7795.2,-7961.1,-8127,-8292.8 -0,-177.09,-354.19,-531.28,-708.38,-885.47,-1062.6,-1239.7,-1416.8,-1593.8,-1770.9,-1948,-2125.1,-2302.2,-2479.3,-2656.4,-2833.5,-3010.6,-3187.7,-3364.8,-3541.9,-3719,-3896.1,-4073.2,-4250.3,-4427.4,-4604.5,-4781.5,-4958.6,-5135.7,-5312.8,-5489.9,-5667,-5844.1,-6021.2,-6198.3,-6375.4,-6552.5,-6729.6,-6906.7,-7083.8,-7260.9,-7438,-7615.1,-7792.1,-7969.2,-8146.3,-8323.4,-8500.5,-8677.6,-8854.7 -0,-187.84,-375.67,-563.51,-751.35,-939.18,-1127,-1314.9,-1502.7,-1690.5,-1878.4,-2066.2,-2254,-2441.9,-2629.7,-2817.5,-3005.4,-3193.2,-3381.1,-3568.9,-3756.7,-3944.6,-4132.4,-4320.2,-4508.1,-4695.9,-4883.7,-5071.6,-5259.4,-5447.3,-5635.1,-5822.9,-6010.8,-6198.6,-6386.4,-6574.3,-6762.1,-6949.9,-7137.8,-7325.6,-7513.5,-7701.3,-7889.1,-8077,-8264.8,-8452.6,-8640.5,-8828.3,-9016.1,-9204,-9391.8 -0,-196.25,-392.49,-588.74,-784.98,-981.23,-1177.5,-1373.7,-1570,-1766.2,-1962.5,-2158.7,-2354.9,-2551.2,-2747.4,-2943.7,-3139.9,-3336.2,-3532.4,-3728.7,-3924.9,-4121.2,-4317.4,-4513.6,-4709.9,-4906.1,-5102.4,-5298.6,-5494.9,-5691.1,-5887.4,-6083.6,-6279.9,-6476.1,-6672.3,-6868.6,-7064.8,-7261.1,-7457.3,-7653.6,-7849.8,-8046.1,-8242.3,-8438.6,-8634.8,-8831,-9027.3,-9223.5,-9419.8,-9616,-9812.3 -0,-199.97,-399.95,-599.92,-799.9,-999.87,-1199.8,-1399.8,-1599.8,-1799.8,-1999.7,-2199.7,-2399.7,-2599.7,-2799.6,-2999.6,-3199.6,-3399.6,-3599.5,-3799.5,-3999.5,-4199.5,-4399.4,-4599.4,-4799.4,-4999.4,-5199.3,-5399.3,-5599.3,-5799.2,-5999.2,-6199.2,-6399.2,-6599.1,-6799.1,-6999.1,-7199.1,-7399,-7599,-7799,-7999,-8198.9,-8398.9,-8598.9,-8798.9,-8998.8,-9198.8,-9398.8,-9598.8,-9798.7,-9998.7 -0,-196.87,-393.74,-590.6,-787.47,-984.34,-1181.2,-1378.1,-1574.9,-1771.8,-1968.7,-2165.5,-2362.4,-2559.3,-2756.2,-2953,-3149.9,-3346.8,-3543.6,-3740.5,-3937.4,-4134.2,-4331.1,-4528,-4724.8,-4921.7,-5118.6,-5315.4,-5512.3,-5709.2,-5906,-6102.9,-6299.8,-6496.6,-6693.5,-6890.4,-7087.2,-7284.1,-7481,-7677.8,-7874.7,-8071.6,-8268.5,-8465.3,-8662.2,-8859.1,-9055.9,-9252.8,-9449.7,-9646.5,-9843.4 -0,-186.02,-372.04,-558.06,-744.08,-930.1,-1116.1,-1302.1 ...(+10776 chars)], aMy=84e-4, bMy=6.2e-4, cMy=1.6e-4, alphaMy=-0.003, betaMy=0.97, QSY1=0.007, QSY2=0, QSY3=0.0015, QSY4=8.5e-05, QSY5=0, QSY6=0, QSY7=0.9, QSY8=-0.4, lam_My=1, VxMy=-20:1:20, FzMy=0:200:1e4, MyMap=[0,1114.7,4367.1,9707.2,17109,26554,38030,51524,67028,84533,1.0403e+05,1.2552e+05,1.4899e+05,1.7444e+05,2.0185e+05,2.3124e+05,2.6259e+05,2.959e+05,3.3117e+05,3.6839e+05,4.0756e+05,4.4868e+05,4.9174e+05,5.3675e+05,5.8369e+05,6.3257e+05,6.8338e+05,7.3613e+05,7.908e+05,8.474e+05,9.0593e+05,9.6638e+05,1.0288e+06,1.093e+06,1.1593e+06,1.2274e+06,1.2974e+06,1.3694e+06,1.4432e+06,1.519e+06,1.5967e+06,1.6763e+06,1.7578e+06,1.8412e+06,1.9265e+06,2.0137e+06,2.1028e+06,2.1938e+06,2.2867e+06,2.3815e+06,2.4782e+06 0,1024.5,4013.8,8921.9,15725,24406,34953,47356,61605,77694,95616,1.1537e+05,1.3694e+05,1.6032e+05,1.8553e+05,2.1254e+05,2.4135e+05,2.7197e+05,3.0438e+05,3.3859e+05,3.7459e+05,4.1238e+05,4.5196e+05,4.9333e+05,5.3647e+05,5.814e+05,6.281e+05,6.7658e+05,7.2683e+05,7.7885e+05,8.3264e+05,8.8821e+05,9.4553e+05,1.0046e+06,1.0655e+06,1.1281e+06,1.1925e+06,1.2586e+06,1.3265e+06,1.3961e+06,1.4675e+06,1.5407e+06,1.6156e+06,1.6922e+06,1.7706e+06,1.8508e+06,1.9327e+06,2.0163e+06,2.1017e+06,2.1889e+06,2.2777e+06 0,938.57,3677,8173.3,14405,22358,32020,43382,56436,71175,87593,1.0568e+05,1.2545e+05,1.4687e+05,1.6996e+05,1.947e+05,2.211e+05,2.4915e+05,2.7884e+05,3.1018e+05,3.4316e+05,3.7778e+05,4.1404e+05,4.5193e+05,4.9146e+05,5.3261e+05,5.754e+05,6.1981e+05,6.6584e+05,7.135e+05,7.6278e+05,8.1368e+05,8.6619e+05,9.2032e+05,9.7607e+05,1.0334e+06,1.0924e+06,1.153e+06,1.2152e+06,1.279e+06,1.3444e+06,1.4114e+06,1.48e+06,1.5502e+06,1.6221e+06,1.6955e+06,1.7705e+06,1.8471e+06,1.9254e+06,2.0052e+06,2.0866e+06 0,856.81,3356.7,7461.3,13151,20411,29231,39603,51520,64974,79962,96478,1.1452e+05,1.3408e+05,1.5515e+05,1.7774e+05,2.0184e+05,2.2744e+05,2.5455e+05,2.8316e+05,3.1327e+05,3.4487e+05,3.7797e+05,4.1256e+05,4.4864e+05,4.8621e+05,5.2527e+05,5.6581e+05,6.0784e+05,6.5134e+05,6.9633e+05,7.4279e+05,7.9073e+05,8.4015e+05,8.9104e+05,9.4341e+05,9.9724e+05,1.0525e+06,1.1093e+06,1.1676e+06,1.2273e+06,1.2885e+06,1.3511e+06,1.4152e+06,1.4808e+06,1.5478e+06,1.6163e+06,1.6862e+06,1.7576e+06,1.8305e+06,1.9048e+06 0,779.25,3052.9,6785.9,11960,18563,26585,36018,46856,59093,72724,87745,1.0415e+05,1.2194e+05,1.4111e+05,1.6165e+05,1.8357e+05,2.0685e+05,2.3151e+05,2.5753e+05,2.8491e+05,3.1365e+05,3.4376e+05,3.7522e+05,4.0803e+05,4.422e+05,4.7772e+05,5.1459e+05,5.5282e+05,5.9238e+05,6.333e+05,6.7556e+05,7.1916e+05,7.641e+05,8.1039e+05,8.5801e+05,9.0697e+05,9.5727e+05,1.0089e+06,1.0619e+06,1.1162e+06,1.1718e+06,1.2288e+06,1.2871e+06,1.3467e+06,1.4077e+06,1.47e+06,1.5336e+06,1.5985e+06,1.6648e+06,1.7324e+06 0,705.9,2765.5,6147.1,10834,16816,24083,32628,42446,53531,65879,79486,94348,1.1046e+05,1.2783e+05,1.4643e+05,1.6629e+05,1.8738e+05,2.0972e+05,2.3329e+05,2.5809e+05,2.8413e+05,3.114e+05,3.399e+05,3.6962e+05,4.0058e+05,4.3276e+05,4.6616e+05,5.0078e+05,5.3662e+05,5.7369e+05,6.1197e+05,6.5146e+05,6.9218e+05,7.3411e+05,7.7725e+05,8.216e+05,8.6717e+05,9.1394e+05,9.6193e+05,1.0111e+06,1.0615e+06,1.1131e+06,1.1659e+06,1.22e+06,1.2752e+06,1.3316e+06,1.3892e+06,1.4481e+06,1.5081e+06,1.5693e+06 0,636.76,2494.6,5545,9773.1,15169,21724,29432,38288,48287,59426,71700,85106,99642,1.153e+05,1.3209e+05,1.5e+05,1.6903e+05,1.8917e+05,2.1044e+05,2.3281e+05,2.563e+05,2.809e+05,3.066e+05,3.3342e+05,3.6134e+05,3.9037e+05,4.205e+05,4.5173e+05,4.8406e+05,5.1749e+05,5.5202e+05,5.8765e+05,6.2438e+05,6.622e+05,7.0111e+05,7.4112e+05,7.8223e+05,8.2442e+05,8.677e+05,9.1208e+05,9.5754e+05,1.0041e+06,1.0517e+06,1.1005e+06,1.1503e+06,1.2012e+06,1.2532e+06,1.3062e+06,1.3604e+06,1.4156e+06 0,571.82,2240.2,4979.5,8776.4,13622,19508,26430,34383,43363,53365,64388,76427,89480,1.0355e+05,1.1862e+05,1.347e+05,1.5179e+05,1.6988e+05,1.8897e+05,2.0907e+05,2.3016e+05,2.5225e+05,2.7534e+05,2.9942e+05,3.2449e+05,3.5056e+05,3.7761e+05,4.0566e+05,4.3469e+05,4.6472e+05,4.9573e+05,5.2772e+05,5.607e+05,5.9467e+05,6.2961e+05,6.6554e+05,7.0245e+05,7.4034e+05,7.7921e+05,8.1906e+05,8.5989e+05,9.017e+05,9.4448e+05,9.8824e+05,1.033e+06,1.0787e+06,1.1254e+06,1.173e+06,1.2216e+06,1.2712e+06 0,511.09,2002.3,4450.7,7844.3,12175,17436 ...(+15095 chars)], Fpl=10, Cr=1e-3, Kt=.008, Tmeas=298.15, Tamb=298.15, extTamb=off, mu_static=0.3, mu_kinetic=0.2, disk_abore=0.05, Rm=0.1778, num_pads=2, drum_abore=0.0508, drum_a=0.123, drum_c=0.212, drum_r=0.15, drum_theta1=0, drum_theta2=126, brake_p_bpt=[1 11.4736842105263 21.9473684210526 32.4210526315789 42.8947368421053 53.3684210526316 63.8421052631579 74.3157894736842 84.7894736842105 95.2631578947368 105.736842105263 116.210526315789 126.684210526316 137.157894736842 147.631578947368 158.105263157895 168.578947368421 179.052631578947 189.526315789474 200], brake_n_bpt=[0 52.6315789473684 105.263157894737 157.894736842105 210.526315789474 263.157894736842 315.789473684211 368.421052631579 421.052631578947 473.684210526316 526.315789473684 578.947368421053 631.578947368421 684.210526315789 736.842105263158 789.473684210526 842.105263157895 894.736842105263 947.368421052632 1000], f_brake_t=[43.4900602404453 42.5056030554862 41.5350898940194 40.5780454442085 39.6340111501808 38.7025443887544 37.7832176914519 36.8756180088306 35.9793460143796 35.0940154454303 34.2192524787115 33.3546951383474 32.4999927342521 31.6548053290159 30.8188032315107 29.991666515561 29.1730845621415 28.362755623661 27.5603864089927 26.765691687993;498.991217495636 487.695866636631 476.560505099801 465.579679307235 454.748127933653 444.060772460445 433.51270824929 423.099196101319 412.81565427025 402.657650900201 392.620896861006 382.701238955775 372.894653477208 363.197240090814 353.605216024701 344.114910546964 334.722759712992 325.425301366216 316.219170376863 307.10109410434;954.492374750826 932.886130217776 911.585920305583 890.581313170261 869.862244717126 849.419000532136 829.242198807128 809.322774193808 789.651962526121 770.221286354971 751.0225412433 732.047782773203 713.289314220164 694.739674852612 676.391628817892 658.238154578366 640.272434863842 622.48784710877 604.877954344734 587.436496520688;1409.99353200602 1378.07639379892 1346.61133551136 1315.58294703329 1284.9763615006 1254.77722860383 1224.97168936497 1195.5463522863 1166.48827078199 1137.78492180974 1109.42418562559 1081.39432659063 1053.68397496312 1026.28210961441 999.178041611083 972.361398609768 945.822110014692 919.550392851325 893.536738312604 867.771898937035;1865.49468926121 1823.26665738007 1781.63675071715 1740.58458089631 1700.09047828407 1660.13545667552 1620.7011799228 1581.76993037878 1543.32457903786 1505.34855726451 1467.82583000789 1430.74087040806 1394.07863570608 1357.82454437621 1321.96445440427 1286.48464264117 1251.37178516554 1216.61293859388 1182.19552228048 1148.10730135338;2320.9958465164 2268.45692096121 2216.66216592293 2165.58621475934 2115.20459506754 2065.49368474721 2016.43067048064 1967.99350847127 1920.16088729373 1872.91219271928 1826.22747439018 1780.08741422549 1734.47329644903 1689.36697913801 1644.75086719747 1600.60788667257 1556.92146031639 1513.67548433643 1470.85430624835 1428.44270376973;2776.49700377159 2713.64718454235 2651.68758112871 2590.58784862237 2530.31871185102 2470.8519128189 2412.16016103848 2354.21708656376 2296.9971955496 2240.47582817405 2184.62911877248 2129.43395804292 2074.86795719199 2020.9094138998 1967.53727999066 1914.73113070398 1862.47113546724 1810.73803007899 1759.51309021622 1708.77810618608;3231.99816102678 3158.8374481235 3086.71299633449 3015.58948248539 2945.43282863449 2876.21014089059 2807.88965159632 2740.44066465625 2673.83350380547 2608.03946362882 2543.03076315477 2478.78050186034 2415.26261793494 2352.4518486616 2290.32369278385 2228.85437473538 2168.02081061809 2107.80057582154 2048.17187418409 1989.11350860242;3687.49931828197 3604.02771170464 3521.73841154027 3440.59111634842 3360.54694541796 3281.56836896228 3203.61914215416 3126.66424274874 3050.66981206134 2975.60309908359 2901.43240753707 2828.12704567777 2755.6572786779 2683.9942834234 2613.11010557704 2542.97761876678 2473.57048576894 2404.8631215641 2336.83065815196 2269.44891101877;4143.00047553716 4049.21797528579 3956.76382674606 3865.59275021144 3775.66106220143 3686.92659703397 3599.34863271199 3512.88782084123 3427.50612031721 3343.16673453836 3259.83405191936 3177.4735894952 3096.05193942085 3015.5367181852 2935.89651837023 2857.10086279818 2779.12016091979 2701.92566730665 2625.48944211983 2549.78431343512;4598.50163279235 4494.40823886693 4391.78924195184 4290.59438407447 4190.77517898491 4092.28482510566 3995.07812326983 3899.11139893372 3804.34242857308 3710.73036999313 3618.23569630166 3526.82013331263 3436.44660016381 3347.079152947 3258.68293116342 3171.22410682959 3084.66983607064 2998.98821304921 2914.1482260877 2830.11971585147;5054.00279004754 4939.59850244808 4826.81465715762 4715.59601793749 4605.88929576838 4497.64305317735 4390.80761382767 4285.3349770262 4181.17873682896 4078.2940054479 3976.63734068395 3876.16667713006 3776.84126090677 3678.62158770879 3581.46934395661 3485.34735086099 ...(+2764 chars)], FNOMIN=2000, lam_Fzo=1, m=10, zo=0, zdoto=0, g=9.81, VERTICAL_STIFFNESS=209000.0, VERTICAL_DAMPING=50, Q_RE0=.99, Q_V1=0, Q_V2=0.047, Q_FZ1=0, Q_FZ2=15.4, Q_FCX=0.134, Q_FCY=.11, Q_CAM=0, PFZ1=0.71, Q_FCY2=-0.48, Q_CAM1=85.2, Q_CAM2=257.0, Q_CAM3=0.512, Q_FYS1=-204500.0, Q_FYS2=-60000, Q_FYS3=88211.7, BOTTOM_OFFST=.01, BOTTOM_STIFF=2000000, zFz=[0 .050 .051], pFz=[10000 1000000], Fzz=[0 1e3 1e4; 0 1e4 1e5], zdotFz=[-20 0 20], Fzzdot=[500 0 -500;250 0 -250], Gndz=0, extGnd=off, FZMIN=0, FZMAX=10000, PRESMIN=10000, PRESMAX=1000000, kappamax=1.5, VXLOW=1, TMIN=0, TMAX=400, blkID=0}
      mask prompts: FxType "autoblks_shared:autoblkLongitudinalWheel:blkPrm_FxType"; rollingType "autoblks_shared:autoblkLongitudinalWheel:blkPrm_rollingType"; BrakeType "autoblks_shared:autoblkLongitudinalWheel:blkPrm_BrakeType"; vertType "autoblks_shared:autoblkLongitudinalWheel:blkPrm_vertType"; lam_x "autoblks_shared:autoblkLongitudinalWheel:blkPrm_lam_x"; extMu "autoblks_shared:autoblkLongitudinalWheel:blkPrm_extMu"; br "autoblks_shared:autoblkLongitudinalWheel:blkPrm_br"; Iyy "autoblks_shared:autoblkLongitudinalWheel:blkPrm_Iyy"; omegao "autoblks_shared:autoblkLongitudinalWheel:blkPrm_omegao"; Lrel "autoblks_shared:autoblkLongitudinalWheel:blkPrm_Lrel"; Re "autoblks_shared:autoblkLongitudinalWheel:blkPrm_Re"; UNLOADED_RADIUS "autoblks_shared:autoblkLongitudinalWheel:blkPrm_UNLOADED_RADIUS"; LONGVL "autoblks_shared:autoblkLongitudinalWheel:blkPrm_LONGVL"; gamma "autoblks_shared:autoblkLongitudinalWheel:blkPrm_gamma"; NOMPRES "autoblks_shared:autoblkLongitudinalWheel:blkPrm_NOMPRES"; press "autoblks_shared:autoblkLongitudinalWheel:blkPrm_press"; extPress "autoblks_shared:autoblkLongitudinalWheel:blkPrm_extPress"; Dx "autoblks_shared:autoblkLongitudinalWheel:blkPrm_Dx"; Cx "autoblks_shared:autoblkLongitudinalWheel:blkPrm_Cx"; Bx "autoblks_shared:autoblkLongitudinalWheel:blkPrm_Bx"; Ex "autoblks_shared:autoblkLongitudinalWheel:blkPrm_Ex"; PCX1 "autoblks_shared:autoblkLongitudinalWheel:blkPrm_PCX1"; PDX1 "autoblks_shared:autoblkLongitudinalWheel:blkPrm_PDX1"; PDX2 "autoblks_shared:autoblkLongitudinalWheel:blkPrm_PDX2"; PDX3 "autoblks_shared:autoblkLongitudinalWheel:blkPrm_PDX3"; PEX1 "autoblks_shared:autoblkLongitudinalWheel:blkPrm_PEX1"; PEX2 "autoblks_shared:autoblkLongitudinalWheel:blkPrm_PEX2"; PEX3 "autoblks_shared:autoblkLongitudinalWheel:blkPrm_PEX3"; PEX4 "autoblks_shared:autoblkLongitudinalWheel:blkPrm_PEX4"; PKX1 "autoblks_shared:autoblkLongitudinalWheel:blkPrm_PKX1"; PKX2 "autoblks_shared:autoblkLongitudinalWheel:blkPrm_PKX2"; PKX3 "autoblks_shared:autoblkLongitudinalWheel:blkPrm_PKX3"; PHX1 "autoblks_shared:autoblkLongitudinalWheel:blkPrm_PHX1"; PHX2 "autoblks_shared:autoblkLongitudinalWheel:blkPrm_PHX2"; PVX1 "autoblks_shared:autoblkLongitudinalWheel:blkPrm_PVX1"; PVX2 "autoblks_shared:autoblkLongitudinalWheel:blkPrm_PVX2"; PPX1 "autoblks_shared:autoblkLongitudinalWheel:blkPrm_PPX1"; PPX2 "autoblks_shared:autoblkLongitudinalWheel:blkPrm_PPX2"; PPX3 "autoblks_shared:autoblkLongitudinalWheel:blkPrm_PPX3"; PPX4 "autoblks_shared:autoblkLongitudinalWheel:blkPrm_PPX4"; lam_muV "autoblks_shared:autoblkLongitudinalWheel:blkPrm_lam_muV"; lam_Kxkappa "autoblks_shared:autoblkLongitudinalWheel:blkPrm_lam_Kxkappa"; lam_Cx "autoblks_shared:autoblkLongitudinalWheel:blkPrm_lam_Cx"; lam_Ex "autoblks_shared:autoblkLongitudinalWheel:blkPrm_lam_Ex"; lam_Hx "autoblks_shared:autoblkLongitudinalWheel:blkPrm_lam_Hx"; lam_Vx "autoblks_shared:autoblkLongitudinalWheel:blkPrm_lam_Vx"; kappaFx "autoblks_shared:autoblkLongitudinalWheel:blkPrm_kappaFx"; FzFx "autoblks_shared:autoblkLongitudinalWheel:blkPrm_FzFx"; FxMap "autoblks_shared:autoblkLongitudinalWheel:blkPrm_FxMap"; aMy "autoblks_shared:autoblkLongitudinalWheel:blkPrm_aMy"; bMy "autoblks_shared:autoblkLongitudinalWheel:blkPrm_bMy"; cMy "autoblks_shared:autoblkLongitudinalWheel:blkPrm_cMy"; alphaMy "autoblks_shared:autoblkLongitudinalWheel:blkPrm_alphaMy"; betaMy "autoblks_shared:autoblkLongitudinalWheel:blkPrm_betaMy"; QSY1 "autoblks_shared:autoblkLongitudinalWheel:blkPrm_QSY1"; QSY2 "autoblks_shared:autoblkLongitudinalWheel:blkPrm_QSY2"; QSY3 "autoblks_shared:autoblkLongitudinalWheel:blkPrm_QSY3"; QSY4 "autoblks_shared:autoblkLongitudinalWheel:blkPrm_QSY4"; QSY5 "autoblks_shared:autoblkLongitudinalWheel:blkPrm_QSY5"; QSY6 "autoblks_shared:autoblkLongitudinalWheel:blkPrm_QSY6"; QSY7 "autoblks_shared:autoblkLongitudinalWheel:blkPrm_QSY7"; QSY8 "autoblks_shared:autoblkLongitudinalWheel:blkPrm_QSY8"; lam_My "autoblks_shared:autoblkLongitudinalWheel:blkPrm_lam_My"; VxMy "autoblks_shared:autoblkLongitudinalWheel:blkPrm_VxMy"; FzMy "autoblks_shared:autoblkLongitudinalWheel:blkPrm_FzMy"; MyMap "autoblks_shared:autoblkLongitudinalWheel:blkPrm_MyMap"; Fpl "autoblks_shared:autoblkLongitudinalWheel:blkPrm_Fpl"; Cr "autoblks_shared:autoblkLongitudinalWheel:blkPrm_Cr"; Kt "autoblks_shared:autoblkLongitudinalWheel:blkPrm_Kt"; Tmeas "autoblks_shared:autoblkLongitudinalWheel:blkPrm_Tmeas"; Tamb "autoblks_shared:autoblkLongitudinalWheel:blkPrm_Tamb"; extTamb "autoblks_shared:autoblkLongitudinalWheel:blkPrm_extTamb"; mu_static "autoblks_shared:autoblkLongitudinalWheel:blkPrm_mu_static"; mu_kinetic "autoblks_shared:autoblkLongitudinalWheel:blkPrm_mu_kinetic"; disk_abore "autoblks_shared:autoblkLongitudinalWheel:blkPrm_disk_abore"; Rm "autoblks_shared:autoblkLongitudinalWheel:blkPrm_Rm"; num_pads "autoblks_shared:autoblkLongitudinalWheel:blkPrm_num_pads"; drum_abore "autoblks_shared:autoblkLongitudinalWheel:blkPrm_drum_abore"; drum_a "autoblks_shared:autoblkLongitudinalWheel:blkPrm_drum_a"; drum_c "autoblks_shared:autoblkLongitudinalWheel:blkPrm_drum_c"; drum_r "autoblks_shared:autoblkLongitudinalWheel:blkPrm_drum_r"; drum_theta1 "autoblks_shared:autoblkLongitudinalWheel:blkPrm_drum_theta1"; drum_theta2 "autoblks_shared:autoblkLongitudinalWheel:blkPrm_drum_theta2"; brake_p_bpt "autoblks_shared:autoblkLongitudinalWheel:blkPrm_brake_p_bpt"; brake_n_bpt "autoblks_shared:autoblkLongitudinalWheel:blkPrm_brake_n_bpt"; f_brake_t "autoblks_shared:autoblkLongitudinalWheel:blkPrm_f_brake_t"; FNOMIN "autoblks_shared:autoblkLongitudinalWheel:blkPrm_FNOMIN"; lam_Fzo "autoblks_shared:autoblkLongitudinalWheel:blkPrm_lam_Fzo"; m "autoblks_shared:autoblkLongitudinalWheel:blkPrm_m"; zo "autoblks_shared:autoblkLongitudinalWheel:blkPrm_zo"; zdoto "autoblks_shared:autoblkLongitudinalWheel:blkPrm_zdoto"; g "autoblks_shared:autoblkLongitudinalWheel:blkPrm_g"; VERTICAL_STIFFNESS "autoblks_shared:autoblkLongitudinalWheel:blkPrm_VERTICAL_STIFFNESS"; VERTICAL_DAMPING "autoblks_shared:autoblkLongitudinalWheel:blkPrm_VERTICAL_DAMPING"; Q_RE0 "autoblks_shared:autoblkLongitudinalWheel:blkPrm_Q_RE0"; Q_V1 "autoblks_shared:autoblkLongitudinalWheel:blkPrm_Q_V1"; Q_V2 "autoblks_shared:autoblkLongitudinalWheel:blkPrm_Q_V2"; Q_FZ1 "autoblks_shared:autoblkLongitudinalWheel:blkPrm_Q_FZ1"; Q_FZ2 "autoblks_shared:autoblkLongitudinalWheel:blkPrm_Q_FZ2"; Q_FCX "autoblks_shared:autoblkLongitudinalWheel:blkPrm_Q_FCX"; Q_FCY "autoblks_shared:autoblkLongitudinalWheel:blkPrm_Q_FCY"; Q_CAM "autoblks_shared:autoblkLongitudinalWheel:blkPrm_Q_CAM"; PFZ1 "autoblks_shared:autoblkLongitudinalWheel:blkPrm_PFZ1"; Q_FCY2 "autoblks_shared:autoblkLongitudinalWheel:blkPrm_Q_FCY2"; Q_CAM1 "autoblks_shared:autoblkLongitudinalWheel:blkPrm_Q_CAM1"; Q_CAM2 "autoblks_shared:autoblkLongitudinalWheel:blkPrm_Q_CAM2"; Q_CAM3 "autoblks_shared:autoblkLongitudinalWheel:blkPrm_Q_CAM3"; Q_FYS1 "autoblks_shared:autoblkLongitudinalWheel:blkPrm_Q_FYS1"; Q_FYS2 "autoblks_shared:autoblkLongitudinalWheel:blkPrm_Q_FYS2"; Q_FYS3 "autoblks_shared:autoblkLongitudinalWheel:blkPrm_Q_FYS3"; BOTTOM_OFFST "autoblks_shared:autoblkLongitudinalWheel:blkPrm_BOTTOM_OFFST"; BOTTOM_STIFF "autoblks_shared:autoblkLongitudinalWheel:blkPrm_BOTTOM_STIFF"; zFz "autoblks_shared:autoblkLongitudinalWheel:blkPrm_zFz"; pFz "autoblks_shared:autoblkLongitudinalWheel:blkPrm_pFz"; Fzz "autoblks_shared:autoblkLongitudinalWheel:blkPrm_Fzz"; zdotFz "autoblks_shared:autoblkLongitudinalWheel:blkPrm_zdotFz"; Fzzdot "autoblks_shared:autoblkLongitudinalWheel:blkPrm_Fzzdot"; Gndz "autoblks_shared:autoblkLongitudinalWheel:blkPrm_Gndz"; extGnd "autoblks_shared:autoblkLongitudinalWheel:blkPrm_extGnd"; FZMIN "autoblks_shared:autoblkLongitudinalWheel:blkPrm_FZMIN"; FZMAX "autoblks_shared:autoblkLongitudinalWheel:blkPrm_FZMAX"; PRESMIN "autoblks_shared:autoblkLongitudinalWheel:blkPrm_PRESMIN"; PRESMAX "autoblks_shared:autoblkLongitudinalWheel:blkPrm_PRESMAX"; kappamax "autoblks_shared:autoblkLongitudinalWheel:blkPrm_kappamax"; VXLOW "autoblks_shared:autoblkLongitudinalWheel:blkPrm_VXLOW"; TMIN "autoblks_shared:autoblkLongitudinalWheel:blkPrm_TMIN"; TMAX "autoblks_shared:autoblkLongitudinalWheel:blkPrm_TMAX"; blkID "autoblks_shared:autoblkLongitudinalWheel:blkPrm_blkID"
      mask help: autoblks_shared:autoblkLongitudinalWheel:blkDesc
      mask init:
      | [~]=autosharedicon('autolibswheel',gcb,0);
      | D = Dx;
      | C = Cx;
      | B = Bx;
      | E = Ex;
      mask Help: eval('autosharedhelp(''pbtirelong'')');
      mask TypeOptions FxType: autoblks_shared:autoblkLongitudinalWheel:blkCmb_FxType_c1 | autoblks_shared:autoblkLongitudinalWheel:blkCmb_FxType_c2 | autoblks_shared:autoblkLongitudinalWheel:blkCmb_FxType_c3
      mask Callback FxType: [~]=autosharedicon('autolibswheel',gcb,5);
      mask TypeOptions rollingType: autoblks_shared:autoblkLongitudinalWheel:blkCmb_rollingType_c1 | autoblks_shared:autoblkLongitudinalWheel:blkCmb_rollingType_c2 | autoblks_shared:autoblkLongitudinalWheel:blkCmb_rollingType_c5 | autoblks_shared:autoblkLongitudinalWheel:blkCmb_rollingType_c3 | autoblks_shared:autoblkLongitudinalWheel:blkCmb_rollingType_c4
      mask Callback rollingType: [~]=autosharedicon('autolibswheel',gcb,2);
      mask TypeOptions BrakeType: autoblks_shared:autoblkLongitudinalWheel:blkCmb_BrakeType_c1 | autoblks_shared:autoblkLongitudinalWheel:blkCmb_BrakeType_c2 | autoblks_shared:autoblkLongitudinalWheel:blkCmb_BrakeType_c3 | autoblks_shared:autoblkLongitudinalWheel:blkCmb_BrakeType_c4
      mask Callback BrakeType: [~]=autosharedicon('autolibswheel',gcb,1);
      mask TypeOptions vertType: autoblks_shared:autoblkLongitudinalWheel:blkCmb_vertType_c1 | autoblks_shared:autoblkLongitudinalWheel:blkCmb_vertType_c2
      mask Callback vertType: [~]=autosharedicon('autolibswheel',gcb,10);
      mask Callback extMu: [~]=autosharedicon('autolibswheel',gcb,9);
      mask Callback extPress: [~]=autosharedicon('autolibswheel',gcb,12);
      mask Callback extTamb: [~]=autosharedicon('autolibswheel',gcb,13);
      mask Callback extGnd: [~]=autosharedicon('autolibswheel',gcb,11);
      mask DialogControl BlockOptions Prompt: autoblks_shared:autoblkLongitudinalWheel:blkDlg_BlockOptions
      mask DialogControl FxType Prompt: Longitudinal Force:
      mask DialogControl rollingType Prompt: Rolling Resistance:
      mask DialogControl BrakeType Prompt: Brake Type:
      mask DialogControl vertType Prompt: Vertical Motion:
      mask DialogControl lam_x Prompt: Longitudinal scaling factor, lam_x []:
      mask DialogControl extMu Prompt: Input friction scale factor
      mask DialogControl wheelParam Prompt: autoblks_shared:autoblkLongitudinalWheel:blkDlg_wheelParam
      mask DialogControl wheelParamPanel Prompt: autoblks_shared:autoblkLongitudinalWheel:blkDlg_wheelParamPanel
      mask DialogControl br Prompt: Axle viscous damping coefficient, br [N*m*s/rad]:
      mask DialogControl Iyy Prompt: Wheel inertia, Iyy [Kg*m^2]:
      mask DialogControl omegao Prompt: Wheel initial angular velocity, omegao [rad/s]:
      mask DialogControl Lrel Prompt: Relaxation length, Lrel [m]:
      mask DialogControl Re Prompt: Loaded radius, Re [m]:
      mask DialogControl UNLOADED_RADIUS Prompt: Unloaded radius, UNLOADED_RADIUS [m]:
      mask DialogControl LONGVL Prompt: Nominal longitudinal speed, LONGVL [m/s]:
      mask DialogControl gamma Prompt: Nominal camber angle, gamma [rad]:
      mask DialogControl NOMPRES Prompt: Nominal inflation pressure, NOMPRES [Pa]:
      mask DialogControl press Prompt: Pressure, press [Pa]:
      mask DialogControl extPress Prompt: Input tire pressure
      mask DialogControl longParamPanel Prompt: autoblks_shared:autoblkLongitudinalWheel:blkDlg_longParamPanel
      mask DialogControl MagicPeakFxParams Prompt: autoblks_shared:autoblkLongitudinalWheel:blkDlg_MagicPeakFxParams
      mask DialogControl Dx Prompt: Pure longitudinal peak factor, Dx []:
      mask DialogControl Cx Prompt: Pure longitudinal shape factor, Cx []:
      mask DialogControl Bx Prompt: Pure longitudinal stiffness factor, Bx []:
      mask DialogControl Ex Prompt: Pure longitudinal curvature factor, Ex []:
      mask DialogControl MagicPureFxoParams Prompt: autoblks_shared:autoblkLongitudinalWheel:blkDlg_MagicPureFxoParams
      mask DialogControl PCX1 Prompt: Cfx shape factor, PCX1 []:
      mask DialogControl PDX1 Prompt: Longitudinal friction at nominal normal load, PDX1 []:
      mask DialogControl PDX2 Prompt: Frictional variation with load, PDX2 []:
      mask DialogControl PDX3 Prompt: Frictional variation with camber, PDX3 [1/rad^2]:
      mask DialogControl PEX1 Prompt: Longitudinal curvature at nominal normal load, PEX1 []:
      mask DialogControl PEX2 Prompt: Variation of curvature factor with load, PEX2 []:
      mask DialogControl PEX3 Prompt: Variation of curvature factor with square of load, PEX3 []:
      mask DialogControl PEX4 Prompt: Longitudinal curvature factor with slip, PEX4 []:
      mask DialogControl PKX1 Prompt: Longitudinal slip stiffness at nominal normal load, PKX1 []:
      mask DialogControl PKX2 Prompt: Variation of slip stiffness with load, PKX2 []:
      mask DialogControl PKX3 Prompt: Slip stiffness exponent factor, PKX3 []:
      mask DialogControl PHX1 Prompt: Horizontal shift in slip ratio at nominal normal load, PHX1 []:
      mask DialogControl PHX2 Prompt: Variation of horizontal slip ratio with load, PHX2 []:
      mask DialogControl PVX1 Prompt: Vertical shift in load at nominal normal load, PVX1 []:
      mask DialogControl PVX2 Prompt: Variation of vertical shift with load, PVX2 []:
      mask DialogControl PPX1 Prompt: Linear variation of longitudinal slip stiffness with tire pressure, PPX1 []:
      mask DialogControl PPX2 Prompt: Quadratic variation of longitudinal slip stiffness with tire pressure, PPX2 []:
      mask DialogControl PPX3 Prompt: Linear variation of peak longitudinal friction with tire pressure, PPX3 []:
      mask DialogControl PPX4 Prompt: Quadratic variation of peak longitudinal friction with tire pressure, PPX4 []:
      mask DialogControl lam_muV Prompt: Slip speed decay function scaling factor, lam_muV []:
      mask DialogControl lam_Kxkappa Prompt: Brake slip stiffness scaling factor, lam_Kxkappa []:
      mask DialogControl lam_Cx Prompt: Longitudinal shape scaling factor, lam_Cx []:
      mask DialogControl lam_Ex Prompt: Longitudinal curvature scaling factor, lam_Ex []:
      mask DialogControl lam_Hx Prompt: Longitudinal horizontal shift scaling factor, lam_Hx []:
      mask DialogControl lam_Vx Prompt: Longitudinal vertical shift scaling factor, lam_Vx []:
      mask DialogControl MappedFxParam Prompt: autoblks_shared:autoblkLongitudinalWheel:blkDlg_MappedFxParam
      mask DialogControl kappaFx Prompt: Slip ratio breakpoints, kappaFx []:
      mask DialogControl FzFx Prompt: Normal force breakpoints, FzFx [N]:
      mask DialogControl FxMap Prompt: Longitudinal force map, FxMap [N]:
      mask DialogControl plotFxMap Prompt: autoblks_shared:autoblkLongitudinalWheel:blkDlg_plotFxMap
      mask DialogControl plotFxMap Callback: [~]=autosharedicon('autolibswheel',gcb,6);
      mask DialogControl rollingParamPanel Prompt: autoblks_shared:autoblkLongitudinalWheel:blkDlg_rollingParamPanel
      mask DialogControl SimpMyParams Prompt: autoblks_shared:autoblkLongitudinalWheel:blkDlg_SimpMyParams
      mask DialogControl aMy Prompt: Velocity independent force coefficient, aMy []:
      mask DialogControl bMy Prompt: Linear velocity force component, bMy [s/m]:
      mask DialogControl cMy Prompt: Quadratic velocity force component, cMy [s^2/m^2]:
      mask DialogControl alphaMy Prompt: Tire pressure exponent, alphaMy []:
      mask DialogControl betaMy Prompt: Normal force exponent, betaMy []:
      mask DialogControl MagicMyParams Prompt: autoblks_shared:autoblkLongitudinalWheel:blkDlg_MagicMyParams
      mask DialogControl QSY1 Prompt: Rolling resistance torque coefficient, QSY1 []:
      mask DialogControl QSY2 Prompt: Longitudinal force rolling resistance coefficient, QSY2 []:
      mask DialogControl QSY3 Prompt: Linear rotational speed rolling resistance coefficient, QSY3 []:
      mask DialogControl QSY4 Prompt: Quartic rotational speed rolling resistance coefficient, QSY4 []:
      mask DialogControl QSY5 Prompt: Camber squared rolling resistance torque, QSY5 [1/rad^2]:
      mask DialogControl QSY6 Prompt: Load based camber squared rolling resistance torque, QSY6 [1/rad^2]:
      mask DialogControl QSY7 Prompt: Normal load rolling resistance coefficient, QSY7 []:
      mask DialogControl QSY8 Prompt: Pressure load rolling resistance coefficient, QSY8 []:
      mask DialogControl lam_My Prompt: Rolling resistance scaling factor, lam_My []:
      mask DialogControl MappedMyParams Prompt: autoblks_shared:autoblkLongitudinalWheel:blkDlg_MappedMyParams
      mask DialogControl VxMy Prompt: Spin axis velocity breakpoints, VxMy [m/s]:
      mask DialogControl FzMy Prompt: Normal force breakpoints, FzMy [N]:
      mask DialogControl MyMap Prompt: Rolling resistance torque map, MyMap [Nm]:
      mask DialogControl plotMyMap Prompt: autoblks_shared:autoblkLongitudinalWheel:blkDlg_plotMyMap
      mask DialogControl plotMyMap Callback: [~]=autosharedicon('autolibswheel',gcb,7);
      mask DialogControl ISOMyParams Prompt: autoblks_shared:autoblkLongitudinalWheel:blkDlg_ISOMyParams
      mask DialogControl Fpl Prompt: Parasitic losses force, Fpl [N]:
      mask DialogControl Cr Prompt: Rolling resistance constant, Cr [N/kN]:
      mask DialogControl Kt Prompt: Thermal correction factor, Kt [1/degC]:
      mask DialogControl Tmeas Prompt: Measured temperature, Tmeas [K]:
      mask DialogControl Tamb Prompt: Ambient temperature, Tamb [K]:
      mask DialogControl extTamb Prompt: Input ambient temperature
      mask DialogControl brakeParamPanel Prompt: autoblks_shared:autoblkLongitudinalWheel:blkDlg_brakeParamPanel
      mask DialogControl GenParams Prompt: autoblks_shared:autoblkLongitudinalWheel:blkDlg_GenParams
      mask DialogControl mu_static Prompt: Static friction coefficient, mu_static []:
      mask DialogControl mu_kinetic Prompt: Kinetic friction coefficient, mu_kinetic []:
      mask DialogControl DiskBrakeParms Prompt: autoblks_shared:autoblkLongitudinalWheel:blkDlg_DiskBrakeParms
      mask DialogControl disk_abore Prompt: Disc brake actuator bore, disk_abore [m]:
      mask DialogControl Rm Prompt: Brake pad mean radius, Rm [m]:
      mask DialogControl num_pads Prompt: Number of brake pads, num_pads []:
      mask DialogControl DrumBrakeParms Prompt: autoblks_shared:autoblkLongitudinalWheel:blkDlg_DrumBrakeParms
      mask DialogControl drum_abore Prompt: Drum brake actuator bore, drum_abore [m]:
      mask DialogControl drum_a Prompt: Shoe pin to drum center distance, drum_a [m]:
      mask DialogControl drum_c Prompt: Shoe pin center to force application point distance, drum_c [m]:
      mask DialogControl drum_r Prompt: Drum internal radius, drum_r [m]:
      mask DialogControl drum_theta1 Prompt: Shoe pin to pad start angle, drum_theta1 [deg]:
      mask DialogControl drum_theta2 Prompt: Shoe pin to pad end angle, drum_theta2 [deg]:
      mask DialogControl MappedBrakeParms Prompt: autoblks_shared:autoblkLongitudinalWheel:blkDlg_MappedBrakeParms
      mask DialogControl brake_p_bpt Prompt: Brake actuator pressure breakpoints, brake_p_bpt [bar]:
      mask DialogControl brake_n_bpt Prompt: Wheel speed breakpoints, brake_n_bpt [rpm]:
      mask DialogControl f_brake_t Prompt: Brake torque map, f_brake_t [Nm]:
      mask DialogControl PlotBrakeTorqueMap Prompt: autoblks_shared:autoblkLongitudinalWheel:blkDlg_PlotBrakeTorqueMap
      mask DialogControl PlotBrakeTorqueMap Callback: [~]=autosharedicon('autolibswheel',gcb,3);
      mask DialogControl vertDynParamPanel Prompt: autoblks_shared:autoblkLongitudinalWheel:blkDlg_vertDynParamPanel
      mask DialogControl FNOMIN Prompt: Nominal normal force, FNOMIN [N]:
      mask DialogControl lam_Fzo Prompt: Nominal rated load scaling factor, lam_Fzo []:
      mask DialogControl m Prompt: Wheel and unsprung mass, m [kg]:
      mask DialogControl zo Prompt: Initial deflection, zo [m]:
      mask DialogControl zdoto Prompt: Initial velocity, zdoto [m/s]:
      mask DialogControl g Prompt: Gravitational acceleration, g [m/s^2]:
      mask DialogControl vertMagicParam Prompt: autoblks_shared:autoblkLongitudinalWheel:blkDlg_vertMagicParam
      mask DialogControl VERTICAL_STIFFNESS Prompt: Vertical tire stiffness, VERTICAL_STIFFNESS [N/m]:
      mask DialogControl VERTICAL_DAMPING Prompt: Vertical tire damping, VERTICAL_DAMPING [N*s/m]:
      mask DialogControl Q_RE0 Prompt: Unloaded to nominal rolling radius ratio, Q_RE0 []:
      mask DialogControl Q_V1 Prompt: Radius rotational speed dependence, Q_V1 []:
      mask DialogControl Q_V2 Prompt: Stiffness rotational speed dependence, Q_V2 []:
      mask DialogControl Q_FZ1 Prompt: Linear load change with deflection, Q_FZ1 []:
      mask DialogControl Q_FZ2 Prompt: Quadratic load change with deflection, Q_FZ2 []:
      mask DialogControl Q_FCX Prompt: Load response to longitudinal force, Q_FCX []:
      mask DialogControl Q_FCY Prompt: Load response to lateral force, Q_FCY []:
      mask DialogControl Q_CAM Prompt: Stiffness response to camber, Q_CAM []:
      mask DialogControl PFZ1 Prompt: Stiffness response to pressure, PFZ1 []:
      mask DialogControl Q_FCY2 Prompt: Load dependent lateral force effect on vertical stiffness, Q_FCY2 []:
      mask DialogControl Q_CAM1 Prompt: Linear load dependent camber angle effect on vertical stiffness, Q_CAM1 []:
      mask DialogControl Q_CAM2 Prompt: Quadratic load dependent camber angle effect on vertical stiffness, Q_CAM2 []:
      mask DialogControl Q_CAM3 Prompt: Linear reduction of stiffness with load and camber angle, Q_CAM3 []:
      mask DialogControl Q_FYS1 Prompt: Constant camber and slip angle on effect on vertical stiffness, Q_FYS1 []:
      mask DialogControl Q_FYS2 Prompt: Linear camber and slip angle on effect on vertical stiffness, Q_FYS2 []:
      mask DialogControl Q_FYS3 Prompt: Quadratic camber and slip angle on effect on vertical stiffness, Q_FYS3 []:
      mask DialogControl BOTTOM_OFFST Prompt: Rim offset distance to bottoming onset, BOTTOM_OFFST [m]:
      mask DialogControl BOTTOM_STIFF Prompt: Vertical stiffness at bottomed tire, BOTTOM_STIFF [N/m]:
      mask DialogControl vertMappedParam Prompt: autoblks_shared:autoblkLongitudinalWheel:blkDlg_vertMappedParam
      mask DialogControl zFz Prompt: Vertical deflection breakpoints, zFz [m]:
      mask DialogControl pFz Prompt: Pressure breakpoints, pFz [Pa]:
      mask DialogControl Fzz Prompt: Force due to deflection, Fzz [N]:
      mask DialogControl zdotFz Prompt: Vertical velocity breakpoints, zdotFz [m/s]:
      mask DialogControl Fzzdot Prompt: Force due to velocity, Fzzdot [N]:
      mask DialogControl Gndz Prompt: Ground displacement, Gndz [m]:
      mask DialogControl extGnd Prompt: Input ground displacement
      mask DialogControl simParamPanel Prompt: autoblks_shared:autoblkLongitudinalWheel:blkDlg_simParamPanel
      mask DialogControl FZMIN Prompt: Minimum normal force, FZMIN [N]:
      mask DialogControl FZMAX Prompt: Maximum normal force, FZMAX [N]:
      mask DialogControl PRESMIN Prompt: Minimum inflation pressure, PRESMIN [Pa]:
      mask DialogControl PRESMAX Prompt: Maximum inflation pressure, PRESMAX [Pa]:
      mask DialogControl kappamax Prompt: Max allowable slip ratio (absolute), kappamax []:
      mask DialogControl VXLOW Prompt: Velocity tolerance used to handle low velocity situations, VXLOW [m/s]:
      mask DialogControl TMIN Prompt: Minimum ambient temperature, TMIN, [K]:
      mask DialogControl TMAX Prompt: Maximum ambient temperature, TMAX [K]:
      mask DialogControl blkID Prompt: Block ID:
      mask Display:
      | try
      |     IconInfo = autosharedicon('autolibswheel', gcb, 8);
      | 
      |     image(IconInfo.image, IconInfo.position);
      | 
      |     for i = 1:numel(IconInfo.lconn)
      |         port_label('lconn', i, IconInfo.lconn{i})
      |     end
      | 
      |     for j = 1:numel(IconInfo.rconn)
      |         port_label('rconn', j, IconInfo.rconn{j})
      |     end
      | 
      |     for k = 1:numel(IconInfo.input)
      |         port_label('input', k, IconInfo.input{k})
      |     end
      | 
      |     for m = 1:numel(IconInfo.output)
      |         port_label('output', m, IconInfo.output{m})
      |     end
      | catch
      |     fprintf('Longitudinal \n Wheel')
      | end
  Vehicle Body 1DOF Longitudinal : Subsystem  VariantControl=SL  mask(Vehicle Body 1DOF Longitudinal){extFMode=off, extMMode=off, extTamb=off, wind3D=off, aMode=aMode, NF=2, NR=2, m=1500, a=1.4, b=1.8, h=.35, Cd=.3, Cl=0, Cpm=0, Af=4, x_o=0, xdot_o=0, Pabs=101325, T=273, g=9.81}
      mask prompts: extFMode "autoblks_shared:autoblkVehBody1Dof:blkPrm_extFMode"; extMMode "autoblks_shared:autoblkVehBody1Dof:blkPrm_extMMode"; extTamb "autoblks_shared:autoblkVehBody1Dof:blkPrm_extTamb"; wind3D "autoblks_shared:autoblkVehBody1Dof:blkPrm_wind3D"; NF "autoblks_shared:autoblkVehBody1Dof:blkPrm_NF"; NR "autoblks_shared:autoblkVehBody1Dof:blkPrm_NR"; m "autoblks_shared:autoblkVehBody1Dof:blkPrm_m"; a "autoblks_shared:autoblkVehBody1Dof:blkPrm_a"; b "autoblks_shared:autoblkVehBody1Dof:blkPrm_b"; h "autoblks_shared:autoblkVehBody1Dof:blkPrm_h"; Cd "autoblks_shared:autoblkVehBody1Dof:blkPrm_Cd"; Cl "autoblks_shared:autoblkVehBody1Dof:blkPrm_Cl"; Cpm "autoblks_shared:autoblkVehBody1Dof:blkPrm_Cpm"; Af "autoblks_shared:autoblkVehBody1Dof:blkPrm_Af"; x_o "autoblks_shared:autoblkVehBody1Dof:blkPrm_x_o"; xdot_o "autoblks_shared:autoblkVehBody1Dof:blkPrm_xdot_o"; Pabs "autoblks_shared:autoblkVehBody1Dof:blkPrm_Pabs"; T "autoblks_shared:autoblkVehBody1Dof:blkPrm_T"; g "autoblks_shared:autoblkVehBody1Dof:blkPrm_g"
      mask help: autoblks_shared:autoblkVehBody1Dof:blkDesc
      mask init:
      | [~]=autosharedicon('autolibvehdyn1dof',gcb,0);
      mask Help: eval('autosharedhelp(''pbvehdyn1dof'')');
      mask Callback extTamb: [~]=autosharedicon('autolibvehdyn1dof',gcb,2);
      mask DialogControl BlockOptions Prompt: autoblks_shared:autoblkVehBody1Dof:blkDlg_BlockOptions
      mask DialogControl extFMode Prompt: External forces
      mask DialogControl extMMode Prompt: External moments
      mask DialogControl extTamb Prompt: Air temperature
      mask DialogControl wind3D Prompt: Wind X,Y,Z components
      mask DialogControl LongPanel Prompt: autoblks_shared:autoblkVehBody1Dof:blkDlg_LongPanel
      mask DialogControl NF Prompt: Number of wheels on front axle, NF [-]:
      mask DialogControl NR Prompt: Number of wheels on rear axle, NR [-]:
      mask DialogControl m Prompt: Mass, m [kg]:
      mask DialogControl a Prompt: Horizontal distance from CG to front axle, a [m]:
      mask DialogControl b Prompt: Horizontal distance from CG to rear axle, b [m]:
      mask DialogControl h Prompt: CG height above axles, h [m]:
      mask DialogControl Cd Prompt: Drag coefficient, Cd [-]:
      mask DialogControl Cl Prompt: Lift coefficient, Cl []:
      mask DialogControl Cpm Prompt: Pitch drag moment coefficient, Cpm []:
      mask DialogControl Af Prompt: Frontal area, Af [m^2]:
      mask DialogControl x_o Prompt: Initial position, x_o [m]:
      mask DialogControl xdot_o Prompt: Initial velocity, xdot_o [m/s]:
      mask DialogControl EnviroPanel Prompt: autoblks_shared:autoblkVehBody1Dof:blkDlg_EnviroPanel
      mask DialogControl Pabs Prompt: Absolute Pressure, Pabs [Pa]:
      mask DialogControl T Prompt: Air Temp, T [K]:
      mask DialogControl g Prompt: Gravitational acceleration, g [m/s^2]:
      mask Display:
      | try
      |     IconInfo = autosharedicon('autolibvehdyn1dof', gcb, 4);
      | 
      |     image(IconInfo.image, IconInfo.position);
      | 
      |     for i = 1:numel(IconInfo.lconn)
      |         port_label('lconn', i, IconInfo.lconn{i})
      |     end
      | 
      |     for j = 1:numel(IconInfo.rconn)
      |         port_label('rconn', j, IconInfo.rconn{j})
      |     end
      | 
      |     for k = 1:numel(IconInfo.input)
      |         port_label('input', k, IconInfo.input{k})
      |     end
      | 
      |     for m = 1:numel(IconInfo.output)
      |         port_label('output', m, IconInfo.output{m})
      |     end
      | catch
      |     fprintf('Vehicle Body \n 1DOF Longitudinal')
      | end
  Vehicle Body 3DOF Longitudinal : Subsystem  VariantControl=SL  mask(Vehicle Body 3DOF Longitudinal){groundType=Grade angle, aMode=aMode, extFMode=off, extMMode=off, extTamb=off, NF=2, NR=2, m=1200, a=1.2, b=1.4, h=.35, Cd=.3, Af=2, x_o=0, xdot_o=0, Cl=.1, z_o=-.35, zdot_o=0, Iyy=3500, Cpm=.1, theta_o=0, q_o=0, FskF=[-50, -1, 0, 2, 3, 52].*200, dzsF=[-5e-3, -1e-4, 0, .2, .2001, .2051], FsbF=[-3e4 -300 -30 0 30 300 3e4], dzdotsF=[-10 -1 -.1 0 .1 1 10], FskR=[-50, -1, 0, 2, 3, 52].*150, dzsR=[-5e-3, -1e-4, 0, .2, .2001, .2051], FsbR=[-3e4 -300 -30 0 30 300 3e4], dzdotsR=[-10 -1 -.1 0 .1 1 10], Pabs=101325, T=273, g=9.81, blkID=0}
      mask prompts: groundType "autoblks_shared:autoblkVehBody3Dof:blkPrm_groundType"; extFMode "autoblks_shared:autoblkVehBody3Dof:blkPrm_extFMode"; extMMode "autoblks_shared:autoblkVehBody3Dof:blkPrm_extMMode"; extTamb "autoblks_shared:autoblkVehBody3Dof:blkPrm_extTamb"; NF "autoblks_shared:autoblkVehBody3Dof:blkPrm_NF"; NR "autoblks_shared:autoblkVehBody3Dof:blkPrm_NR"; m "autoblks_shared:autoblkVehBody3Dof:blkPrm_m"; a "autoblks_shared:autoblkVehBody3Dof:blkPrm_a"; b "autoblks_shared:autoblkVehBody3Dof:blkPrm_b"; h "autoblks_shared:autoblkVehBody3Dof:blkPrm_h"; Cd "autoblks_shared:autoblkVehBody3Dof:blkPrm_Cd"; Af "autoblks_shared:autoblkVehBody3Dof:blkPrm_Af"; x_o "autoblks_shared:autoblkVehBody3Dof:blkPrm_x_o"; xdot_o "autoblks_shared:autoblkVehBody3Dof:blkPrm_xdot_o"; Cl "autoblks_shared:autoblkVehBody3Dof:blkPrm_Cl"; z_o "autoblks_shared:autoblkVehBody3Dof:blkPrm_z_o"; zdot_o "autoblks_shared:autoblkVehBody3Dof:blkPrm_zdot_o"; Iyy "autoblks_shared:autoblkVehBody3Dof:blkPrm_Iyy"; Cpm "autoblks_shared:autoblkVehBody3Dof:blkPrm_Cpm"; theta_o "autoblks_shared:autoblkVehBody3Dof:blkPrm_theta_o"; q_o "autoblks_shared:autoblkVehBody3Dof:blkPrm_q_o"; FskF "autoblks_shared:autoblkVehBody3Dof:blkPrm_FskF"; dzsF "autoblks_shared:autoblkVehBody3Dof:blkPrm_dzsF"; FsbF "autoblks_shared:autoblkVehBody3Dof:blkPrm_FsbF"; dzdotsF "autoblks_shared:autoblkVehBody3Dof:blkPrm_dzdotsF"; FskR "autoblks_shared:autoblkVehBody3Dof:blkPrm_FskR"; dzsR "autoblks_shared:autoblkVehBody3Dof:blkPrm_dzsR"; FsbR "autoblks_shared:autoblkVehBody3Dof:blkPrm_FsbR"; dzdotsR "autoblks_shared:autoblkVehBody3Dof:blkPrm_dzdotsR"; Pabs "autoblks_shared:autoblkVehBody3Dof:blkPrm_Pabs"; T "autoblks_shared:autoblkVehBody3Dof:blkPrm_T"; g "autoblks_shared:autoblkVehBody3Dof:blkPrm_g"; blkID "autoblks_shared:autoblkVehBody3Dof:blkPrm_blkID"
      mask help: autoblks_shared:autoblkVehBody3Dof:blkDesc
      mask init:
      | [~]=autosharedicon('autolibvehdyn3dof',gcb,0);
      mask Help: eval('autosharedhelp(''pbvehdyn3dof'')');
      mask TypeOptions groundType: autoblks_shared:autoblkVehBody3Dof:blkCmb_groundTypeGradeangle | autoblks_shared:autoblkVehBody3Dof:blkCmb_groundTypeAxledisplacementvelocity | autoblks_shared:autoblkVehBody3Dof:blkCmb_groundTypeExternalsuspension
      mask Callback groundType: [~]=autosharedicon('autolibvehdyn3dof',gcb,2);
      mask Callback extTamb: [~]=autosharedicon('autolibvehdyn3dof',gcb,4);
      mask DialogControl BlockOptions Prompt: autoblks_shared:autoblkVehBody3Dof:blkDlg_BlockOptions
      mask DialogControl groundType Prompt: Ground interaction type:
      mask DialogControl extFMode Prompt: External forces
      mask DialogControl extMMode Prompt: External moments
      mask DialogControl extTamb Prompt: Air temperature
      mask DialogControl VehParm Prompt: autoblks_shared:autoblkVehBody3Dof:blkDlg_VehParm
      mask DialogControl LongPanel Prompt: autoblks_shared:autoblkVehBody3Dof:blkDlg_LongPanel
      mask DialogControl NF Prompt: Number of wheels on front axle, NF []:
      mask DialogControl NR Prompt: Number of wheels on rear axle, NR []:
      mask DialogControl m Prompt: Mass, m [kg]:
      mask DialogControl a Prompt: Horizontal distance from CG to front axle, a [m]:
      mask DialogControl b Prompt: Horizontal distance from CG to rear axle, b [m]:
      mask DialogControl h Prompt: CG height above axles, h [m]:
      mask DialogControl Cd Prompt: Drag coefficient, Cd []:
      mask DialogControl Af Prompt: Frontal area, Af [m^2]:
      mask DialogControl x_o Prompt: Initial position, x_o [m]:
      mask DialogControl xdot_o Prompt: Initial velocity, xdot_o [m/s]:
      mask DialogControl VertPanel Prompt: autoblks_shared:autoblkVehBody3Dof:blkDlg_VertPanel
      mask DialogControl Cl Prompt: Lift coefficient, Cl []:
      mask DialogControl z_o Prompt: Initial vertical position, z_o [m]:
      mask DialogControl zdot_o Prompt: Initial vertical velocity, zdot_o [m/s]:
      mask DialogControl PitchParam Prompt: autoblks_shared:autoblkVehBody3Dof:blkDlg_PitchParam
      mask DialogControl Iyy Prompt: Inertia, Iyy [kg*m^2]:
      mask DialogControl Cpm Prompt: Pitch drag moment coefficient, Cpm []:
      mask DialogControl theta_o Prompt: Initial pitch angle, theta_o [rad]:
      mask DialogControl q_o Prompt: Initial angular velocity, q_o [rad/s]:
      mask DialogControl SuspGroup Prompt: autoblks_shared:autoblkVehBody3Dof:blkDlg_SuspGroup
      mask DialogControl SuspPanel Prompt: autoblks_shared:autoblkVehBody3Dof:blkDlg_SuspPanel
      mask DialogControl FskF Prompt: Front axle stiffness force data, FskF [N]:
      mask DialogControl dzsF Prompt: Front axle displacement data, dzsF [m]:
      mask DialogControl FsbF Prompt: Front axle damping force data, FsbF [N]:
      mask DialogControl dzdotsF Prompt: Front axle velocity data, dzdotsF [m/s]:
      mask DialogControl FskR Prompt: Rear axle stiffness force data, FskR [N]:
      mask DialogControl dzsR Prompt: Rear axle displacement data, dzsR [m]:
      mask DialogControl FsbR Prompt: Rear axle damping  force data, FsbR [N]:
      mask DialogControl dzdotsR Prompt: Rear axle velocity data, dzdotsR [m/s]:
      mask DialogControl SuspPlot Prompt: autoblks_shared:autoblkVehBody3Dof:blkDlg_SuspPlot
      mask DialogControl SuspPlot Callback: [~]=autosharedicon('autolibvehdyn3dof',gcb,3);
      mask DialogControl EnviroPanel Prompt: autoblks_shared:autoblkVehBody3Dof:blkDlg_EnviroPanel
      mask DialogControl Pabs Prompt: Absolute Pressure, Pabs [Pa]:
      mask DialogControl T Prompt: Air Temp, T [K]:
      mask DialogControl g Prompt: Gravitational acceleration, g [m/s^2]:
      mask DialogControl blkID Prompt: block ID:
      mask Display:
      | try
      |     IconInfo = autosharedicon('autolibvehdyn3dof', gcb, 5);
      | 
      |     image(IconInfo.image, IconInfo.position);
      | 
      |     for i = 1:numel(IconInfo.lconn)
      |         port_label('lconn', i, IconInfo.lconn{i})
      |     end
      | 
      |     for j = 1:numel(IconInfo.rconn)
      |         port_label('rconn', j, IconInfo.rconn{j})
      |     end
      | 
      |     for k = 1:numel(IconInfo.input)
      |         port_label('input', k, IconInfo.input{k})
      |     end
      | 
      |     for m = 1:numel(IconInfo.output)
      |         port_label('output', m, IconInfo.output{m})
      |     end
      | catch
      |     fprintf('Vehicle Body \n 3DOF Longitudinal')
      | end
  Vehicle Body 3DOF Single Track : Subsystem  mask(Vehicle Body 3DOF Lateral){trackMode=Dual, inputMode=External longitudinal forces, frontSteerMode=on, rearSteerMode=off, windMode=off, muMode=off, extFMode=off, extMMode=off, extXo=off, extpsio=off, extxdoto=off, extro=off, extYo=off, extTamb=off, extydoto=off, aMode=aMode, NF=2, NR=2, m=2000, a=1.4, b=1.6, h=0.35, X_o=0, xdot_o=0, CalphaMode=off, sigmaMode=off, d=0, w=[1.4,1.4], Cy_f=12e3, Cy_r=11e3, sigma_f=.1, sigma_r=.1, alpha_f_brk=[-.1 .1], Cy_f_data=[-9e3 9e3], alpha_r_brk=[-.1 .1], Cy_r_data=[-9e3 9e3], Y_o=0, ydot_o=0, Izz=4000, psi_o=0, r_o=0, Af=2, Cd=.3, Cl=.1, Cpm=.1, beta_w=[0:0.01:0.3], Cs=[0:0.03:0.9], Cym=[0:0.01:0.3], Pabs=101325, Tair=273, g=9.81, mu=1, xdot_tol=.01, Fznom=5000, Fxtire_sat=1e6, Fytire_sat=1e6, longOff=0, latOff=0, vertOff=0, wrapAng=off}
      mask prompts: trackMode "autoblks_shared:autoblkVehBody3DofLat:blkPrm_trackMode"; inputMode "autoblks_shared:autoblkVehBody3DofLat:blkPrm_inputMode"; frontSteerMode "autoblks_shared:autoblkVehBody3DofLat:blkPrm_frontSteerMode"; rearSteerMode "autoblks_shared:autoblkVehBody3DofLat:blkPrm_rearSteerMode"; windMode "autoblks_shared:autoblkVehBody3DofLat:blkPrm_windMode"; muMode "autoblks_shared:autoblkVehBody3DofLat:blkPrm_muMode"; extFMode "autoblks_shared:autoblkVehBody3DofLat:blkPrm_extFMode"; extMMode "autoblks_shared:autoblkVehBody3DofLat:blkPrm_extMMode"; extXo "autoblks_shared:autoblkVehBody3DofLat:blkPrm_extXo"; extpsio "autoblks_shared:autoblkVehBody3DofLat:blkPrm_extpsio"; extxdoto "autoblks_shared:autoblkVehBody3DofLat:blkPrm_extxdoto"; extro "autoblks_shared:autoblkVehBody3DofLat:blkPrm_extro"; extYo "autoblks_shared:autoblkVehBody3DofLat:blkPrm_extYo"; extTamb "autoblks_shared:autoblkVehBody3DofLat:blkPrm_extTamb"; extydoto "autoblks_shared:autoblkVehBody3DofLat:blkPrm_extydoto"; NF "autoblks_shared:autoblkVehBody3DofLat:blkPrm_NF"; NR "autoblks_shared:autoblkVehBody3DofLat:blkPrm_NR"; m "autoblks_shared:autoblkVehBody3DofLat:blkPrm_m"; a "autoblks_shared:autoblkVehBody3DofLat:blkPrm_a"; b "autoblks_shared:autoblkVehBody3DofLat:blkPrm_b"; h "autoblks_shared:autoblkVehBody3DofLat:blkPrm_h"; X_o "autoblks_shared:autoblkVehBody3DofLat:blkPrm_X_o"; xdot_o "autoblks_shared:autoblkVehBody3DofLat:blkPrm_xdot_o"; CalphaMode "autoblks_shared:autoblkVehBody3DofLat:blkPrm_CalphaMode"; sigmaMode "autoblks_shared:autoblkVehBody3DofLat:blkPrm_sigmaMode"; d "autoblks_shared:autoblkVehBody3DofLat:blkPrm_d"; w "autoblks_shared:autoblkVehBody3DofLat:blkPrm_w"; Cy_f "autoblks_shared:autoblkVehBody3DofLat:blkPrm_Cy_f"; Cy_r "autoblks_shared:autoblkVehBody3DofLat:blkPrm_Cy_r"; sigma_f "autoblks_shared:autoblkVehBody3DofLat:blkPrm_sigma_f"; sigma_r "autoblks_shared:autoblkVehBody3DofLat:blkPrm_sigma_r"; alpha_f_brk "autoblks_shared:autoblkVehBody3DofLat:blkPrm_alpha_f_brk"; Cy_f_data "autoblks_shared:autoblkVehBody3DofLat:blkPrm_Cy_f_data"; alpha_r_brk "autoblks_shared:autoblkVehBody3DofLat:blkPrm_alpha_r_brk"; Cy_r_data "autoblks_shared:autoblkVehBody3DofLat:blkPrm_Cy_r_data"; Y_o "autoblks_shared:autoblkVehBody3DofLat:blkPrm_Y_o"; ydot_o "autoblks_shared:autoblkVehBody3DofLat:blkPrm_ydot_o"; Izz "autoblks_shared:autoblkVehBody3DofLat:blkPrm_Izz"; psi_o "autoblks_shared:autoblkVehBody3DofLat:blkPrm_psi_o"; r_o "autoblks_shared:autoblkVehBody3DofLat:blkPrm_r_o"; Af "autoblks_shared:autoblkVehBody3DofLat:blkPrm_Af"; Cd "autoblks_shared:autoblkVehBody3DofLat:blkPrm_Cd"; Cl "autoblks_shared:autoblkVehBody3DofLat:blkPrm_Cl"; Cpm "autoblks_shared:autoblkVehBody3DofLat:blkPrm_Cpm"; beta_w "autoblks_shared:autoblkVehBody3DofLat:blkPrm_beta_w"; Cs "autoblks_shared:autoblkVehBody3DofLat:blkPrm_Cs"; Cym "autoblks_shared:autoblkVehBody3DofLat:blkPrm_Cym"; Pabs "autoblks_shared:autoblkVehBody3DofLat:blkPrm_Pabs"; Tair "autoblks_shared:autoblkVehBody3DofLat:blkPrm_Tair"; g "autoblks_shared:autoblkVehBody3DofLat:blkPrm_g"; mu "autoblks_shared:autoblkVehBody3DofLat:blkPrm_mu"; xdot_tol "autoblks_shared:autoblkVehBody3DofLat:blkPrm_xdot_tol"; Fznom "autoblks_shared:autoblkVehBody3DofLat:blkPrm_Fznom"; Fxtire_sat "autoblks_shared:autoblkVehBody3DofLat:blkPrm_Fxtire_sat"; Fytire_sat "autoblks_shared:autoblkVehBody3DofLat:blkPrm_Fytire_sat"; longOff "autoblks_shared:autoblkVehBody3DofLat:blkPrm_longOff"; latOff "autoblks_shared:autoblkVehBody3DofLat:blkPrm_latOff"; vertOff "autoblks_shared:autoblkVehBody3DofLat:blkPrm_vertOff"; wrapAng "autoblks_shared:autoblkVehBody3DofLat:blkPrm_wrapAng"
      mask help: autoblks_shared:autoblkVehBody3DofLat:blkDesc
      mask init:
      | [~]=autosharedicon('vehdynliblat3dof',gcb,0);
      mask Help: eval('autosharedhelp(''vb3doflat'')');
      mask TypeOptions trackMode: autoblks_shared:autoblkVehBody3DofLat:blkCmb_trackMode_c1 | autoblks_shared:autoblkVehBody3DofLat:blkCmb_trackMode_c2
      mask Callback trackMode: [~]=autosharedicon('vehdynliblat3dof',gcb,5);
      mask TypeOptions inputMode: autoblks_shared:autoblkVehBody3DofLat:blkCmb_inputMode_c1 | autoblks_shared:autoblkVehBody3DofLat:blkCmb_inputMode_c2 | autoblks_shared:autoblkVehBody3DofLat:blkCmb_inputMode_c3
      mask Callback inputMode: [~]=autosharedicon('vehdynliblat3dof',gcb,1);
      mask Callback muMode: [~]=autosharedicon('vehdynliblat3dof',gcb,2);
      mask Callback extXo: [~]=autosharedicon('vehdynliblat3dof',gcb,7);
      mask Callback extpsio: [~]=autosharedicon('vehdynliblat3dof',gcb,7);
      mask Callback extxdoto: [~]=autosharedicon('vehdynliblat3dof',gcb,7);
      mask Callback extro: [~]=autosharedicon('vehdynliblat3dof',gcb,7);
      mask Callback extYo: [~]=autosharedicon('vehdynliblat3dof',gcb,7);
      mask Callback extTamb: [~]=autosharedicon('vehdynliblat3dof',gcb,6);
      mask Callback extydoto: [~]=autosharedicon('vehdynliblat3dof',gcb,7);
      mask Callback CalphaMode: [~]=autosharedicon('vehdynliblat3dof',gcb,3);
      mask Callback sigmaMode: [~]=autosharedicon('vehdynliblat3dof',gcb,4);
      mask DialogControl blockConfig Prompt: autoblks_shared:autoblkVehBody3DofLat:blkDlg_blockConfig
      mask DialogControl trackMode Prompt: Vehicle track:
      mask DialogControl inputMode Prompt: Axle forces:
      mask DialogControl extModePanel Prompt: autoblks_shared:autoblkVehBody3DofLat:blkDlg_extModePanel
      mask DialogControl frontSteerMode Prompt: Front wheel steering
      mask DialogControl rearSteerMode Prompt: Rear wheel steering
      mask DialogControl windMode Prompt: External wind
      mask DialogControl muMode Prompt: External friction
      mask DialogControl extFMode Prompt: External forces
      mask DialogControl extMMode Prompt: External moments
      mask DialogControl extXo Prompt: Initial longitudinal position
      mask DialogControl extpsio Prompt: Initial yaw angle
      mask DialogControl extxdoto Prompt: Initial longitudinal velocity
      mask DialogControl extro Prompt: Initial yaw rate
      mask DialogControl extYo Prompt: Initial lateral position
      mask DialogControl extTamb Prompt: Air temperature
      mask DialogControl extydoto Prompt: Initial lateral velocity
      mask DialogControl ParameterGroupVar Prompt: autoblks_shared:autoblkVehBody3DofLat:blkDlg_ParameterGroupVar
      mask DialogControl LongPanel Prompt: autoblks_shared:autoblkVehBody3DofLat:blkDlg_LongPanel
      mask DialogControl NF Prompt: Number of wheels on front axle, NF [-]:
      mask DialogControl NR Prompt: Number of wheels on rear axle, NR [-]:
      mask DialogControl m Prompt: Vehicle mass, m [kg]:
      mask DialogControl a Prompt: Longitudinal distance from center of mass to front axle, a [m]:
      mask DialogControl b Prompt: Longitudinal distance from center of mass to rear axle, b [m]:
      mask DialogControl h Prompt: Vertical distance from center of mass to axle plane, h [m]:
      mask DialogControl X_o Prompt: Initial inertial frame longitudinal position, X_o [m]:
      mask DialogControl xdot_o Prompt: Initial longitudinal velocity, xdot_o [m/s]:
      mask DialogControl LatPanel Prompt: autoblks_shared:autoblkVehBody3DofLat:blkDlg_LatPanel
      mask DialogControl CalphaMode Prompt: Mapped corner stiffness:
      mask DialogControl sigmaMode Prompt: Include relaxation length dynamics:
      mask DialogControl d Prompt: Lateral distance from geometric centerline to center of mass, d [m]:
      mask DialogControl w Prompt: Track width, w [m]:
      mask DialogControl Cy_f Prompt: Front tire corner stiffness, Cy_f [N/rad]:
      mask DialogControl Cy_r Prompt: Rear tire axle corner stiffness, Cy_r [N/rad]:
      mask DialogControl sigma_f Prompt: Front tire(s) relaxation length, sigma_f [m]:
      mask DialogControl sigma_r Prompt: Rear tire(s) relaxation length, sigma_r [m]:
      mask DialogControl alpha_f_brk Prompt: Front axle slip angle breakpoints, alpha_f_brk [rad]:
      mask DialogControl Cy_f_data Prompt: Front axle corner data, Cy_f_data [N/rad]:
      mask DialogControl alpha_r_brk Prompt: Rear axle slip angle breakpoints, alpha_r_brk [rad]:
      mask DialogControl Cy_r_data Prompt: Rear axle corner data, Cy_r_data [N/rad]:
      mask DialogControl Y_o Prompt: Initial inertial frame lateral displacement, Y_o [m]:
      mask DialogControl ydot_o Prompt: Initial lateral velocity, ydot_o [m/s]:
      mask DialogControl YawPanel Prompt: autoblks_shared:autoblkVehBody3DofLat:blkDlg_YawPanel
      mask DialogControl Izz Prompt: Yaw polar inertia, Izz [kg*m^2]:
      mask DialogControl psi_o Prompt: Initial yaw angle, psi_o [rad]:
      mask DialogControl r_o Prompt: Initial yaw rate, r_o [rad/s]:
      mask DialogControl AeroParams Prompt: autoblks_shared:autoblkVehBody3DofLat:blkDlg_AeroParams
      mask DialogControl Af Prompt: Longitudinal drag area, Af [m^2]:
      mask DialogControl Cd Prompt: Longitudinal drag coefficient, Cd [-]:
      mask DialogControl Cl Prompt: Longitudinal lift coefficient, Cl [-]:
      mask DialogControl Cpm Prompt: Longitudinal drag pitch moment, Cpm [-]:
      mask DialogControl beta_w Prompt: Relative wind angle vector, beta_w [rad]:
      mask DialogControl Cs Prompt: Side force coefficient vector, Cs [-]:
      mask DialogControl Cym Prompt: Yaw moment coefficient vector, Cym [-]:
      mask DialogControl EnviroPanel Prompt: autoblks_shared:autoblkVehBody3DofLat:blkDlg_EnviroPanel
      mask DialogControl Pabs Prompt: Absolute pressure, Pabs [Pa]:
      mask DialogControl Tair Prompt: Air temperature, Tair [K]:
      mask DialogControl g Prompt: Gravitational acceleration, g [m/s^2]:
      mask DialogControl mu Prompt: Nominal friction scaling factor, mu [-]:
      mask DialogControl SimPanel Prompt: autoblks_shared:autoblkVehBody3DofLat:blkDlg_SimPanel
      mask DialogControl xdot_tol Prompt: Longitudinal velocity tolerance, xdot_tol [m/s]:
      mask DialogControl Fznom Prompt: Nominal normal force, Fznom [N]:
      mask DialogControl Fxtire_sat Prompt: Longitudinal force limit, Fxtire_sat [N]:
      mask DialogControl Fytire_sat Prompt: Lateral force limit, Fytire_sat [N]:
      mask DialogControl longOff Prompt: Geometric longitudinal offset from axle plane, longOff [m]:
      mask DialogControl latOff Prompt: Geometric lateral offset from center plane, latOff [m]:
      mask DialogControl vertOff Prompt: Geometric vertical offset from axle plane, vertOff [m]:
      mask DialogControl wrapAng Prompt: Wrap Euler angles, wrapAng
      mask Display:
      | try
      |     IconInfo = autosharedicon('vehdynliblat3dof',gcb,8);
      | 
      |     image(IconInfo.image, IconInfo.position);
      | 
      |     for i = 1:numel(IconInfo.lconn)
      |         port_label('lconn', i, IconInfo.lconn{i})
      |     end
      | 
      |     for j = 1:numel(IconInfo.rconn)
      |         port_label('rconn', j, IconInfo.rconn{j})
      |     end
      | 
      |     for k = 1:numel(IconInfo.input)
      |         port_label('input', k, IconInfo.input{k})
      |     end
      | 
      |     for m = 1:numel(IconInfo.output)
      |         port_label('output', m, IconInfo.output{m})
      |     end
      | catch
      |     fprintf('Vehicle Body \n 3DOF Lateral')
      | end
  Vehicle Body Total Road Load : Subsystem  VariantControl=SL1dof  mask(Vehicle Body Total Road Load){input_type=Force, aMode=aMode, m=1200, a=196, b=2.232, c=0.389, g=9.81, x_o=0, xdot_o=0}
      mask prompts: input_type "autoblks_shared:autoblkVehBodyTotalRoadLoad:blkPrm_input_type"; m "autoblks_shared:autoblkVehBodyTotalRoadLoad:blkPrm_m"; a "autoblks_shared:autoblkVehBodyTotalRoadLoad:blkPrm_a"; b "autoblks_shared:autoblkVehBodyTotalRoadLoad:blkPrm_b"; c "autoblks_shared:autoblkVehBodyTotalRoadLoad:blkPrm_c"; g "autoblks_shared:autoblkVehBodyTotalRoadLoad:blkPrm_g"; x_o "autoblks_shared:autoblkVehBodyTotalRoadLoad:blkPrm_x_o"; xdot_o "autoblks_shared:autoblkVehBodyTotalRoadLoad:blkPrm_xdot_o"
      mask help: autoblks_shared:autoblkVehBodyTotalRoadLoad:blkDesc
      mask init:
      | [~]=autosharedicon('autolibvehdyncdt',gcb,0);
      mask Help: eval('autosharedhelp(''pbvehdyncdt'')');
      mask TypeOptions input_type: autoblks_shared:autoblkVehBodyTotalRoadLoad:blkCmb_input_typeForce | autoblks_shared:autoblkVehBodyTotalRoadLoad:blkCmb_input_typePower | autoblks_shared:autoblkVehBodyTotalRoadLoad:blkCmb_input_typeKinematic
      mask DialogControl BlockOptions Prompt: autoblks_shared:autoblkVehBodyTotalRoadLoad:blkDlg_BlockOptions
      mask DialogControl input_type Prompt: Input Mode:
      mask DialogControl m Prompt: Mass, m [kg]:
      mask DialogControl a Prompt: Rolling resistance coefficient, a [N]:
      mask DialogControl b Prompt: Rolling and driveline resistance coefficient, b [N*s/m]:
      mask DialogControl c Prompt: Aerodynamic drag coefficient, c [N*s^2/m^2]:
      mask DialogControl g Prompt: Gravitational constant, g [m/s^2]:
      mask DialogControl x_o Prompt: Initial position, x_o [m]:
      mask DialogControl xdot_o Prompt: Initial velocity, xdot_o [m/s]:
      mask Display:
      | try
      |     IconInfo = autosharedicon('autolibvehdyncdt', gcb, 4);
      | 
      |     image(IconInfo.image, IconInfo.position);
      | 
      |     for i = 1:numel(IconInfo.lconn)
      |         port_label('lconn', i, IconInfo.lconn{i})
      |     end
      | 
      |     for j = 1:numel(IconInfo.rconn)
      |         port_label('rconn', j, IconInfo.rconn{j})
      |     end
      | 
      |     for k = 1:numel(IconInfo.input)
      |         port_label('input', k, IconInfo.input{k})
      |     end
      | 
      |     for m = 1:numel(IconInfo.output)
      |         port_label('output', m, IconInfo.output{m})
      |     end
      | catch
      |     fprintf('Vehicle Body \n Total Road Load')
      | end
